simulink model "ConSys_A1"  (Simulink 8.3)
settings: Solver=ode3  StartTime=0.0  StopTime=Time(end)  FixedStep=Ts  RelTol=1e-3
values from neighbouring files (symbols this model uses):
  d = r*h    (= 1.6)    [StartUp_A1.m]
  d0 = d*h    (= 0.0032)    [StartUp_A1.m]
  h = 0.002    [StartUp_A1.m]
  Ka = diag([ 3  20  20  150  355  520])    [StartUp_A1.m]
  Kd = diag([ 3   5  25  100   15 1050])    [StartUp_A1.m]
  Ki = diag([35 555 810 7410 1850 5815])    [StartUp_A1.m]
  Kp = diag([55 180 350 1960  680 4450])    [StartUp_A1.m]
  r = 800    [StartUp_A1.m]
  TD = ss(Atd,Btd,Ctd,Dtd,Ts)    [StartUp_A1.m]
  Ts = 1/200    (= 0.005)    [StartUp_A1.m]
undefined symbols (not defined in the file or in its folder): DiscIntNeverNeededParam
undefined symbols (not defined in the file): ADAMS_cwd, ADAMS_exec, ADAMS_host, ADAMS_init, ADAMS_inputs, ADAMS_outputs, ADAMS_prefix, ADAMS_static, ADAMS_sysdir
libraries: cstblocks x6
(part 8 of 9)

== matlab function A2/MATLAB Function 5 ==
  data: q input double; V5 output double; dq input double
function V5 = V5(q,dq)
%#codegen
Th1=q(1,1); Th2=q(2,1); Th3=q(3,1); Th4=q(4,1); Th5=q(5,1); Th6=q(6,1);
dTh1=dq(1); dTh2=dq(2); dTh3=dq(3); dTh4=dq(4); dTh5=dq(5); dTh6=dq(6);
%---------------------------
V511=(0.5*(sin(Th2 + Th3)*cos(Th5) + cos(Th2 + Th3)*cos(Th4)*sin(Th5))*(4.0e-6*cos(Th6)*(sin(Th2 + Th3)*cos(Th5) + cos(Th2 + Th3)*cos(Th4)*sin(Th5)) + 0.000116*sin(Th2 + Th3)*sin(Th5) - 0.000116*cos(Th2 + Th3)*cos(Th4)*cos(Th5)) - 0.5*(cos(Th6)*(sin(Th2 + Th3)*sin(Th5) - 1.0*cos(Th2 + Th3)*cos(Th4)*cos(Th5)) + cos(Th2 + Th3)*sin(Th4)*sin(Th6))*(0.001043*cos(Th6)*(sin(Th2 + Th3)*cos(Th5) + cos(Th2 + Th3)*cos(Th4)*sin(Th5)) + 4.0e-6*sin(Th2 + Th3)*sin(Th5) - 4.0e-6*cos(Th2 + Th3)*cos(Th4)*cos(Th5)) - 0.5*(sin(Th2 + Th3)*sin(Th5) - 1.0*cos(Th2 + Th3)*cos(Th4)*cos(Th5))*(4.0e-6*cos(Th6)*(sin(Th2 + Th3)*sin(Th5) - 1.0*cos(Th2 + Th3)*cos(Th4)*cos(Th5)) - 0.000116*sin(Th2 + Th3)*cos(Th5) - 0.000116*cos(Th2 + Th3)*cos(Th4)*sin(Th5) + 4.0e-6*cos(Th2 + Th3)*sin(Th4)*sin(Th6)) - 1.0*(0.000115*cos(Th6)*(sin(Th5)*(sin(Th1)*sin(Th4) - 1.0*sin(Th2 + Th3)*cos(Th1)*cos(Th4)) + cos(Th2 + Th3)*cos(Th1)*cos(Th5)) + 0.02603*cos(Th5)*(sin(Th1)*sin(Th4) - 1.0*sin(Th2 + Th3)*cos(Th1)*cos(Th4)) - 0.02603*cos(Th2 + Th3)*cos(Th1)*sin(Th5))*(0.07*cos(Th1) + 0.05206*sin(Th5)*(sin(Th1)*sin(Th4) - 1.0*sin(Th2 + Th3)*cos(Th1)*cos(Th4)) + 0.126*cos(Th2 + Th3)*cos(Th1) - 0.00023*sin(Th6)*(cos(Th4)*sin(Th1) + sin(Th2 + Th3)*cos(Th1)*sin(Th4)) - 0.36*cos(Th1)*sin(Th2) - 0.00023*cos(Th6)*(cos(Th5)*(sin(Th1)*sin(Th4) - 1.0*sin(Th2 + Th3)*cos(Th1)*cos(Th4)) - 1.0*cos(Th2 + Th3)*cos(Th1)*sin(Th5)) + 0.05206*cos(Th2 + Th3)*cos(Th1)*cos(Th5) + 0.254*cos(Th1)*cos(Th2)*cos(Th3) - 0.254*cos(Th1)*sin(Th2)*sin(Th3)) + (0.00152*cos(Th5)*(cos(Th1)*sin(Th4) + sin(Th2 + Th3)*cos(Th4)*sin(Th1)) + 0.00002*sin(Th5)*(cos(Th1)*sin(Th4) + sin(Th2 + Th3)*cos(Th4)*sin(Th1)) - 0.00002*cos(Th2 + Th3)*cos(Th5)*sin(Th1) + 0.00152*cos(Th2 + Th3)*sin(Th1)*sin(Th5))*(0.00002*cos(Th5)*(cos(Th1)*sin(Th4) + sin(Th2 + Th3)*cos(Th4)*sin(Th1)) - 0.126*cos(Th2 + Th3)*sin(Th1) - 0.07*sin(Th1) - 0.00152*sin(Th5)*(cos(Th1)*sin(Th4) + sin(Th2 + Th3)*cos(Th4)*sin(Th1)) - 0.00062*cos(Th1)*cos(Th4) + 0.36*sin(Th1)*sin(Th2) + 0.00152*cos(Th2 + Th3)*cos(Th5)*sin(Th1) + 0.00002*cos(Th2 + Th3)*sin(Th1)*sin(Th5) + 0.00062*sin(Th2 + Th3)*sin(Th1)*sin(Th4) - 0.254*cos(Th2)*cos(Th3)*sin(Th1) + 0.254*sin(Th1)*sin(Th2)*sin(Th3)) - 1.0*(0.00152*cos(Th5)*(sin(Th1)*sin(Th4) - 1.0*sin(Th2 + Th3)*cos(Th1)*cos(Th4)) + 0.00002*sin(Th5)*(sin(Th1)*sin(Th4) - 1.0*sin(Th2 + Th3)*cos(Th1)*cos(Th4)) + 0.00002*cos(Th2 + Th3)*cos(Th1)*cos(Th5) - 0.00152*cos(Th2 + Th3)*cos(Th1)*sin(Th5))*(0.00152*sin(Th5)*(sin(Th1)*sin(Th4) - 1.0*sin(Th2 + Th3)*cos(Th1)*cos(Th4)) - 0.00002*cos(Th5)*(sin(Th1)*sin(Th4) - 1.0*sin(Th2 + Th3)*cos(Th1)*cos(Th4)) - 0.07*cos(Th1) - 0.126*cos(Th2 + Th3)*cos(Th1) + 0.36*cos(Th1)*sin(Th2) + 0.00062*cos(Th4)*sin(Th1) + 0.00152*cos(Th2 + Th3)*cos(Th1)*cos(Th5) + 0.00002*cos(Th2 + Th3)*cos(Th1)*sin(Th5) + 0.00062*sin(Th2 + Th3)*cos(Th1)*sin(Th4) - 0.254*cos(Th1)*cos(Th2)*cos(Th3) + 0.254*cos(Th1)*sin(Th2)*sin(Th3)) + (0.000115*cos(Th6)*(sin(Th5)*(cos(Th1)*sin(Th4) + sin(Th2 + Th3)*cos(Th4)*sin(Th1)) - 1.0*cos(Th2 + Th3)*cos(Th5)*sin(Th1)) + 0.02603*cos(Th5)*(cos(Th1)*sin(Th4) + sin(Th2 + Th3)*cos(Th4)*sin(Th1)) + 0.02603*cos(Th2 + Th3)*sin(Th1)*sin(Th5))*(0.07*sin(Th1) + 0.00023*sin(Th6)*(cos(Th1)*cos(Th4) - 1.0*sin(Th2 + Th3)*sin(Th1)*sin(Th4)) + 0.00023*cos(Th6)*(cos(Th5)*(cos(Th1)*sin(Th4) + sin(Th2 + Th3)*cos(Th4)*sin(Th1)) + cos(Th2 + Th3)*sin(Th1)*sin(Th5)) + 0.126*cos(Th2 + Th3)*sin(Th1) - 0.05206*sin(Th5)*(cos(Th1)*sin(Th4) + sin(Th2 + Th3)*cos(Th4)*sin(Th1)) - 0.36*sin(Th1)*sin(Th2) + 0.05206*cos(Th2 + Th3)*cos(Th5)*sin(Th1) + 0.254*cos(Th2)*cos(Th3)*sin(Th1) - 0.254*sin(Th1)*sin(Th2)*sin(Th3)) - 0.5*cos(Th6)*(sin(Th2 + Th3)*cos(Th5) + cos(Th2 + Th3)*cos(Th4)*sin(Th5))*(0.001043*cos(Th6)*(sin(Th2 + Th3)*sin(Th5) - 1.0*cos(Th2 + Th3)*cos(Th4)*cos(Th5)) - 4.0e-6*sin(Th2 + Th3)*cos(Th5) - 4.0e-6*cos(Th2 + Th3)*cos(Th4)*sin(Th5) + 0.001043*cos(Th2 + Th3)*sin(Th4)*sin(Th6)) - 0.5*sin(Th6)*(sin(Th2 + Th3)*cos(Th5) + cos(Th2 + Th3)*cos(Th4)*sin(Th5))*(0.00104*sin(Th6)*(sin(Th2 + Th3)*sin(Th5) - 1.0*cos(Th2 + Th3)*cos(Th4)*cos(Th5)) - 0.00104*cos(Th2 + Th3)*cos(Th6)*sin(Th4)) - 0.004409*sin(Th2 + Th3)^2*cos(Th5)*sin(Th5) - 0.00052*sin(Th6)*(sin(Th2 + Th3)*cos(Th5) + cos(Th2 + Th3)*cos(Th4)*sin(Th5))*(sin(Th6)*(sin(Th2 + Th3)*sin(Th5) - 1.0*cos(Th2 + Th3)*cos(Th4)*cos(Th5)) - 1.0*cos(Th2 + Th3)*cos(Th6)*sin(Th4)) + 0.004409*cos(Th2 + Th3)*sin(Th2 + Th3)*cos(Th4)*cos(Th5)^2 - 0.004409*cos(Th2 + Th3)*sin(Th2 + Th3)*cos(Th4)*sin(Th5)^2 + 0.00004*cos(Th2 + Th3)^2*cos(Th4)*cos(Th5)*sin(Th4) + 0.004409*cos(Th2 + Th3)^2*cos(Th4)^2*cos(Th5)*sin(Th5) - 0.00004*cos(Th2 + Th3)*sin(Th2 + Th3)*sin(Th4)*sin(Th5))*dTh1*dTh1;
V512=(0.000058586*cos(Th2)*cos(Th3)*cos(Th5) - 1.86e-8*cos(Th2)*cos(Th3)*sin(Th5) + 0.013235*cos(Th2)*cos(Th5)*sin(Th4) + 0.0042472*cos(Th2)*sin(Th3)*sin(Th4) + 0.0042472*cos(Th3)*sin(Th2)*sin(Th4) - 0.000058586*cos(Th5)*sin(Th2)*sin(Th3) - 0.0000108*cos(Th2)*sin(Th4)*sin(Th5) + 1.86e-8*sin(Th2)*sin(Th3)*sin(Th5) + 3.04e-8*cos(Th2)*cos(Th3)*cos(Th4)*sin(Th4) - 6.2e-9*cos(Th2)*cos(Th4)*cos(Th5)*sin(Th3) - 6.2e-9*cos(Th3)*cos(Th4)*cos(Th5)*sin(Th2) + 0.00001498*cos(Th2)*cos(Th3)*cos(Th5)*sin(Th6) - 0.000019529*cos(Th2)*cos(Th4)*sin(Th3)*sin(Th5) + 0.013971*cos(Th2)*cos(Th5)*sin(Th3)*sin(Th4) - 0.000019529*cos(Th3)*cos(Th4)*sin(Th2)*sin(Th5) + 0.013971*cos(Th3)*cos(Th5)*sin(Th2)*sin(Th4) + 0.0000621*cos(Th2)*cos(Th6)*sin(Th4)*sin(Th5) - 3.04e-8*cos(Th4)*sin(Th2)*sin(Th3)*sin(Th4) - 0.0000114*cos(Th2)*sin(Th3)*sin(Th4)*sin(Th5) - 0.0000114*cos(Th3)*sin(Th2)*sin(Th4)*sin(Th5) - 0.00001498*cos(Th5)*sin(Th2)*sin(Th3)*sin(Th6) - 0.000039058*cos(Th2)*cos(Th3)*cos(Th4)^2*cos(Th5) + 1.24e-8*cos(Th2)*cos(Th3)*cos(Th4)^2*sin(Th5) + 0.0066904*cos(Th2)*cos(Th5)^2*sin(Th3)*sin(Th4) + 0.0066904*cos(Th3)*cos(Th5)^2*sin(Th2)*sin(Th4) + 0.000039058*cos(Th4)^2*cos(Th5)*sin(Th2)*sin(Th3) - 4.4603e-6*cos(Th2)*cos(Th6)^2*sin(Th3)*sin(Th4) - 4.4603e-6*cos(Th3)*cos(Th6)^2*sin(Th2)*sin(Th4) - 1.24e-8*cos(Th4)^2*sin(Th2)*sin(Th3)*sin(Th5) + 9.9869e-6*cos(Th2)*cos(Th3)*cos(Th4)*cos(Th6)*sin(Th4) - 4.4603e-6*cos(Th2)*cos(Th3)*cos(Th6)*sin(Th5)*sin(Th6) + 6.08e-8*cos(Th2)*cos(Th5)*sin(Th3)*sin(Th4)*sin(Th5) + 6.08e-8*cos(Th3)*cos(Th5)*sin(Th2)*sin(Th4)*sin(Th5) - 9.9869e-6*cos(Th4)*cos(Th6)*sin(Th2)*sin(Th3)*sin(Th4) - 4.9934e-6*cos(Th2)*cos(Th4)*sin(Th3)*sin(Th5)*sin(Th6) + 0.00006555*cos(Th2)*cos(Th6)*sin(Th3)*sin(Th4)*sin(Th5) - 4.9934e-6*cos(Th3)*cos(Th4)*sin(Th2)*sin(Th5)*sin(Th6) + 0.00006555*cos(Th3)*cos(Th6)*sin(Th2)*sin(Th4)*sin(Th5) + 4.4603e-6*cos(Th6)*sin(Th2)*sin(Th3)*sin(Th5)*sin(Th6) - 6.08e-8*cos(Th2)*cos(Th3)*cos(Th4)*cos(Th5)^2*sin(Th4) - 9.9869e-6*cos(Th2)*cos(Th3)*cos(Th4)^2*cos(Th5)*sin(Th6) + 6.08e-8*cos(Th4)*cos(Th5)^2*sin(Th2)*sin(Th3)*sin(Th4) + 9.9869e-6*cos(Th4)^2*cos(Th5)*sin(Th2)*sin(Th3)*sin(Th6) + 2.9736e-6*cos(Th2)*cos(Th5)^2*cos(Th6)^2*sin(Th3)*sin(Th4) + 2.9736e-6*cos(Th3)*cos(Th5)^2*cos(Th6)^2*sin(Th2)*sin(Th4) - 0.000019974*cos(Th2)*cos(Th3)*cos(Th4)*cos(Th5)^2*cos(Th6)*sin(Th4) + 2.9736e-6*cos(Th2)*cos(Th3)*cos(Th4)^2*cos(Th6)*sin(Th5)*sin(Th6) + 0.000019974*cos(Th4)*cos(Th5)^2*cos(Th6)*sin(Th2)*sin(Th3)*sin(Th4) - 2.9736e-6*cos(Th4)^2*cos(Th6)*sin(Th2)*sin(Th3)*sin(Th5)*sin(Th6) + 0.0066904*cos(Th2)*cos(Th3)*cos(Th4)*cos(Th5)*sin(Th4)*sin(Th5) - 1.4868e-6*cos(Th2)*cos(Th4)*cos(Th5)*cos(Th6)*sin(Th3)*sin(Th6) - 1.4868e-6*cos(Th3)*cos(Th4)*cos(Th5)*cos(Th6)*sin(Th2)*sin(Th6) + 0.000019974*cos(Th2)*cos(Th5)*cos(Th6)*sin(Th3)*sin(Th4)*sin(Th5) + 0.000019974*cos(Th3)*cos(Th5)*cos(Th6)*sin(Th2)*sin(Th4)*sin(Th5) - 0.0066904*cos(Th4)*cos(Th5)*sin(Th2)*sin(Th3)*sin(Th4)*sin(Th5) - 2.9736e-6*cos(Th4)*cos(Th5)*cos(Th6)^2*sin(Th2)*sin(Th3)*sin(Th4)*sin(Th5) + 2.9736e-6*cos(Th2)*cos(Th3)*cos(Th4)*cos(Th5)*cos(Th6)^2*sin(Th4)*sin(Th5))*dTh1*dTh2;
V513=(0.000058586*cos(Th2)*cos(Th3)*cos(Th5) - 1.86e-8*cos(Th2)*cos(Th3)*sin(Th5) + 0.0042472*cos(Th2)*sin(Th3)*sin(Th4) + 0.0042472*cos(Th3)*sin(Th2)*sin(Th4) - 0.000058586*cos(Th5)*sin(Th2)*sin(Th3) + 1.86e-8*sin(Th2)*sin(Th3)*sin(Th5) + 3.04e-8*cos(Th2)*cos(Th3)*cos(Th4)*sin(Th4) - 6.2e-9*cos(Th2)*cos(Th4)*cos(Th5)*sin(Th3) - 6.2e-9*cos(Th3)*cos(Th4)*cos(Th5)*sin(Th2) + 0.00001498*cos(Th2)*cos(Th3)*cos(Th5)*sin(Th6) - 0.000019529*cos(Th2)*cos(Th4)*sin(Th3)*sin(Th5) + 0.013971*cos(Th2)*cos(Th5)*sin(Th3)*sin(Th4) - 0.000019529*cos(Th3)*cos(Th4)*sin(Th2)*sin(Th5) + 0.013971*cos(Th3)*cos(Th5)*sin(Th2)*sin(Th4) - 3.04e-8*cos(Th4)*sin(Th2)*sin(Th3)*sin(Th4) - 0.0000114*cos(Th2)*sin(Th3)*sin(Th4)*sin(Th5) - 0.0000114*cos(Th3)*sin(Th2)*sin(Th4)*sin(Th5) - 0.00001498*cos(Th5)*sin(Th2)*sin(Th3)*sin(Th6) - 0.000039058*cos(Th2)*cos(Th3)*cos(Th4)^2*cos(Th5) + 1.24e-8*cos(Th2)*cos(Th3)*cos(Th4)^2*sin(Th5) + 0.0066904*cos(Th2)*cos(Th5)^2*sin(Th3)*sin(Th4) + 0.0066904*cos(Th3)*cos(Th5)^2*sin(Th2)*sin(Th4) + 0.000039058*cos(Th4)^2*cos(Th5)*sin(Th2)*sin(Th3) - 4.4603e-6*cos(Th2)*cos(Th6)^2*sin(Th3)*sin(Th4) - 4.4603e-6*cos(Th3)*cos(Th6)^2*sin(Th2)*sin(Th4) - 1.24e-8*cos(Th4)^2*sin(Th2)*sin(Th3)*sin(Th5) + 9.9869e-6*cos(Th2)*cos(Th3)*cos(Th4)*cos(Th6)*sin(Th4) - 4.4603e-6*cos(Th2)*cos(Th3)*cos(Th6)*sin(Th5)*sin(Th6) + 6.08e-8*cos(Th2)*cos(Th5)*sin(Th3)*sin(Th4)*sin(Th5) + 6.08e-8*cos(Th3)*cos(Th5)*sin(Th2)*sin(Th4)*sin(Th5) - 9.9869e-6*cos(Th4)*cos(Th6)*sin(Th2)*sin(Th3)*sin(Th4) - 4.9934e-6*cos(Th2)*cos(Th4)*sin(Th3)*sin(Th5)*sin(Th6) + 0.00006555*cos(Th2)*cos(Th6)*sin(Th3)*sin(Th4)*sin(Th5) - 4.9934e-6*cos(Th3)*cos(Th4)*sin(Th2)*sin(Th5)*sin(Th6) + 0.00006555*cos(Th3)*cos(Th6)*sin(Th2)*sin(Th4)*sin(Th5) + 4.4603e-6*cos(Th6)*sin(Th2)*sin(Th3)*sin(Th5)*sin(Th6) - 6.08e-8*cos(Th2)*cos(Th3)*cos(Th4)*cos(Th5)^2*sin(Th4) - 9.9869e-6*cos(Th2)*cos(Th3)*cos(Th4)^2*cos(Th5)*sin(Th6) + 6.08e-8*cos(Th4)*cos(Th5)^2*sin(Th2)*sin(Th3)*sin(Th4) + 9.9869e-6*cos(Th4)^2*cos(Th5)*sin(Th2)*sin(Th3)*sin(Th6) + 2.9736e-6*cos(Th2)*cos(Th5)^2*cos(Th6)^2*sin(Th3)*sin(Th4) + 2.9736e-6*cos(Th3)*cos(Th5)^2*cos(Th6)^2*sin(Th2)*sin(Th4) - 0.000019974*cos(Th2)*cos(Th3)*cos(Th4)*cos(Th5)^2*cos(Th6)*sin(Th4) + 2.9736e-6*cos(Th2)*cos(Th3)*cos(Th4)^2*cos(Th6)*sin(Th5)*sin(Th6) + 0.000019974*cos(Th4)*cos(Th5)^2*cos(Th6)*sin(Th2)*sin(Th3)*sin(Th4) - 2.9736e-6*cos(Th4)^2*cos(Th6)*sin(Th2)*sin(Th3)*sin(Th5)*sin(Th6) + 0.0066904*cos(Th2)*cos(Th3)*cos(Th4)*cos(Th5)*sin(Th4)*sin(Th5) - 1.4868e-6*cos(Th2)*cos(Th4)*cos(Th5)*cos(Th6)*sin(Th3)*sin(Th6) - 1.4868e-6*cos(Th3)*cos(Th4)*cos(Th5)*cos(Th6)*sin(Th2)*sin(Th6) + 0.000019974*cos(Th2)*cos(Th5)*cos(Th6)*sin(Th3)*sin(Th4)*sin(Th5) + 0.000019974*cos(Th3)*cos(Th5)*cos(Th6)*sin(Th2)*sin(Th4)*sin(Th5) - 0.0066904*cos(Th4)*cos(Th5)*sin(Th2)*sin(Th3)*sin(Th4)*sin(Th5) - 2.9736e-6*cos(Th4)*cos(Th5)*cos(Th6)^2*sin(Th2)*sin(Th3)*sin(Th4)*sin(Th5) + 2.9736e-6*cos(Th2)*cos(Th3)*cos(Th4)*cos(Th5)*cos(Th6)^2*sin(Th4)*sin(Th5))*dTh1*dTh3;
V514=(7.0e-7*cos(Th4)*sin(Th5) - 3.04e-8*cos(Th2)*sin(Th3) - 3.04e-8*cos(Th3)*sin(Th2) - 0.00085785*cos(Th4)*cos(Th5) - 0.010938*cos(Th2)*cos(Th3)*cos(Th4) - 9.9869e-6*cos(Th2)*cos(Th6)*sin(Th3) - 9.9869e-6*cos(Th3)*cos(Th6)*sin(Th2) + 0.0044118*cos(Th4)*cos(Th5)*sin(Th2) - 4.025e-6*cos(Th4)*cos(Th6)*sin(Th5) + 0.010938*cos(Th4)*sin(Th2)*sin(Th3) - 3.6e-6*cos(Th4)*sin(Th2)*sin(Th5) + 6.08e-8*cos(Th2)*cos(Th5)^2*sin(Th3) + 6.08e-8*cos(Th3)*cos(Th5)^2*sin(Th2) - 0.0046569*cos(Th2)*cos(Th3)*cos(Th4)*cos(Th5) + 3.8e-6*cos(Th2)*cos(Th3)*cos(Th4)*sin(Th5) - 1.86e-8*cos(Th2)*cos(Th3)*cos(Th5)*sin(Th4) - 0.000058586*cos(Th2)*cos(Th3)*sin(Th4)*sin(Th5) + 0.0046569*cos(Th4)*cos(Th5)*sin(Th2)*sin(Th3) - 0.0066904*cos(Th2)*cos(Th5)*sin(Th3)*sin(Th5) - 0.0066904*cos(Th3)*cos(Th5)*sin(Th2)*sin(Th5) + 0.0000207*cos(Th4)*cos(Th6)*sin(Th2)*sin(Th5) - 3.8e-6*cos(Th4)*sin(Th2)*sin(Th3)*sin(Th5) + 1.86e-8*cos(Th5)*sin(Th2)*sin(Th3)*sin(Th4) + 0.000058586*sin(Th2)*sin(Th3)*sin(Th4)*sin(Th5) + 0.0066904*cos(Th2)*cos(Th3)*cos(Th4)*cos(Th5)^2 + 1.4868e-6*cos(Th2)*cos(Th3)*cos(Th4)*cos(Th6)^2 + 0.000019974*cos(Th2)*cos(Th5)^2*cos(Th6)*sin(Th3) + 0.000019974*cos(Th3)*cos(Th5)^2*cos(Th6)*sin(Th2) - 0.0066904*cos(Th4)*cos(Th5)^2*sin(Th2)*sin(Th3) - 1.4868e-6*cos(Th4)*cos(Th6)^2*sin(Th2)*sin(Th3) + 6.08e-8*cos(Th2)*cos(Th3)*cos(Th4)*cos(Th5)*sin(Th5) - 0.00002185*cos(Th2)*cos(Th3)*cos(Th4)*cos(Th6)*sin(Th5) - 6.08e-8*cos(Th4)*cos(Th5)*sin(Th2)*sin(Th3)*sin(Th5) - 0.00001498*cos(Th2)*cos(Th3)*sin(Th4)*sin(Th5)*sin(Th6) + 0.00002185*cos(Th4)*cos(Th6)*sin(Th2)*sin(Th3)*sin(Th5) + 0.00001498*sin(Th2)*sin(Th3)*sin(Th4)*sin(Th5)*sin(Th6) - 2.9736e-6*cos(Th2)*cos(Th5)*cos(Th6)^2*sin(Th3)*sin(Th5) - 2.9736e-6*cos(Th3)*cos(Th5)*cos(Th6)^2*sin(Th2)*sin(Th5) + 2.9736e-6*cos(Th2)*cos(Th3)*cos(Th4)*cos(Th5)^2*cos(Th6)^2 - 2.9736e-6*cos(Th4)*cos(Th5)^2*cos(Th6)^2*sin(Th2)*sin(Th3) + 0.000019974*cos(Th2)*cos(Th3)*cos(Th4)*cos(Th5)*cos(Th6)*sin(Th5) - 4.4603e-6*cos(Th2)*cos(Th3)*cos(Th5)*cos(Th6)*sin(Th4)*sin(Th6) - 0.000019974*cos(Th4)*cos(Th5)*cos(Th6)*sin(Th2)*sin(Th3)*sin(Th5) + 4.4603e-6*cos(Th5)*cos(Th6)*sin(Th2)*sin(Th3)*sin(Th4)*sin(Th6))*dTh1*dTh4;
V515=(7.0e-7*cos(Th5)*sin(Th4) + 0.00085785*sin(Th4)*sin(Th5) - 6.2e-9*cos(Th2)*cos(Th5)*sin(Th3) - 6.2e-9*cos(Th3)*cos(Th5)*sin(Th2) - 4.025e-6*cos(Th5)*cos(Th6)*sin(Th4) - 0.000019529*cos(Th2)*sin(Th3)*sin(Th5) - 0.000019529*cos(Th3)*sin(Th2)*sin(Th5) - 3.6e-6*cos(Th5)*sin(Th2)*sin(Th4) - 0.0044118*sin(Th2)*sin(Th4)*sin(Th5) + 0.000019529*cos(Th2)*cos(Th3)*cos(Th4)*cos(Th5) - 6.2e-9*cos(Th2)*cos(Th3)*cos(Th4)*sin(Th5) + 3.8e-6*cos(Th2)*cos(Th3)*cos(Th5)*sin(Th4) + 0.0046569*cos(Th2)*cos(Th3)*sin(Th4)*sin(Th5) - 0.000019529*cos(Th4)*cos(Th5)*sin(Th2)*sin(Th3) + 0.0000207*cos(Th5)*cos(Th6)*sin(Th2)*sin(Th4) + 6.2e-9*cos(Th4)*sin(Th2)*sin(Th3)*sin(Th5) - 3.8e-6*cos(Th5)*sin(Th2)*sin(Th3)*sin(Th4) - 4.9934e-6*cos(Th2)*sin(Th3)*sin(Th5)*sin(Th6) - 4.9934e-6*cos(Th3)*sin(Th2)*sin(Th5)*sin(Th6) - 0.0046569*sin(Th2)*sin(Th3)*sin(Th4)*sin(Th5) + 4.9934e-6*cos(Th2)*cos(Th3)*cos(Th4)*cos(Th5)*sin(Th6) - 0.00002185*cos(Th2)*cos(Th3)*cos(Th5)*cos(Th6)*sin(Th4) - 1.4868e-6*cos(Th2)*cos(Th5)*cos(Th6)*sin(Th3)*sin(Th6) - 1.4868e-6*cos(Th3)*cos(Th5)*cos(Th6)*sin(Th2)*sin(Th6) - 4.9934e-6*cos(Th4)*cos(Th5)*sin(Th2)*sin(Th3)*sin(Th6) + 0.00002185*cos(Th5)*cos(Th6)*sin(Th2)*sin(Th3)*sin(Th4) - 1.4868e-6*cos(Th2)*cos(Th3)*cos(Th4)*cos(Th6)*sin(Th5)*sin(Th6) + 1.4868e-6*cos(Th4)*cos(Th6)*sin(Th2)*sin(Th3)*sin(Th5)*sin(Th6))*dTh1*dTh5;
V516=(0.000060987*cos(Th2)*sin(Th3)*sin(Th5) + 0.000060987*cos(Th3)*sin(Th2)*sin(Th5) + 4.025e-6*sin(Th4)*sin(Th5)*sin(Th6) - 0.000060987*cos(Th2)*cos(Th3)*cos(Th4)*cos(Th5) + 0.00001498*cos(Th2)*cos(Th5)*cos(Th6)*sin(Th3) + 0.00001498*cos(Th3)*cos(Th5)*cos(Th6)*sin(Th2) + 0.000060987*cos(Th4)*cos(Th5)*sin(Th2)*sin(Th3) - 0.0000207*sin(Th2)*sin(Th4)*sin(Th5)*sin(Th6) - 5.9471e-6*cos(Th2)*cos(Th6)^2*sin(Th3)*sin(Th5) - 5.9471e-6*cos(Th3)*cos(Th6)^2*sin(Th2)*sin(Th5) + 0.00001498*cos(Th2)*cos(Th3)*cos(Th4)*cos(Th6)*sin(Th5) - 5.9471e-6*cos(Th2)*cos(Th3)*cos(Th6)*sin(Th4)*sin(Th6) + 0.00002185*cos(Th2)*cos(Th3)*sin(Th4)*sin(Th5)*sin(Th6) - 0.00001498*cos(Th4)*cos(Th6)*sin(Th2)*sin(Th3)*sin(Th5) + 5.9471e-6*cos(Th6)*sin(Th2)*sin(Th3)*sin(Th4)*sin(Th6) - 0.00002185*sin(Th2)*sin(Th3)*sin(Th4)*sin(Th5)*sin(Th6) + 5.9471e-6*cos(Th2)*cos(Th3)*cos(Th4)*cos(Th5)*cos(Th6)^2 - 5.9471e-6*cos(Th4)*cos(Th5)*cos(Th6)^2*sin(Th2)*sin(Th3))*dTh1*dTh6;
%---------------------------
V521=(0.00002*cos(Th2 + Th3)*cos(Th5) - 0.0026665*sin(Th2 + Th3)*sin(Th4) + 6.2e-9*sin(Th2 + Th3)*cos(Th4)*cos(Th5) + 2.0e-6*cos(Th2 + Th3)*cos(Th5)*sin(Th6) + 0.000019529*sin(Th2 + Th3)*cos(Th4)*sin(Th5) + 0.0015441*sin(Th2 + Th3)*cos(Th5)*sin(Th4) - 1.26e-6*sin(Th2 + Th3)*sin(Th4)*sin(Th5) + 0.0044118*cos(Th2)*cos(Th5)*sin(Th4) - 0.000039529*cos(Th2 + Th3)*cos(Th4)^2*cos(Th5) - 3.6e-6*cos(Th2)*sin(Th4)*sin(Th5) - 4.712e-7*cos(Th2 + Th3)*cos(Th5)*sin(Th4)^2 + 6.2e-9*cos(Th2 + Th3)*cos(Th4)^2*sin(Th5) - 6.2e-9*cos(Th2 + Th3)*sin(Th4)^2*sin(Th5) + 0.0060117*sin(Th2 + Th3)*cos(Th5)^2*sin(Th4) - 1.5e-6*sin(Th2 + Th3)*cos(Th6)^2*sin(Th4) - 0.00067872*sin(Th2 + Th3)*sin(Th4)*sin(Th5)^2 + 4.0e-6*cos(Th2 + Th3)*cos(Th4)*cos(Th6)*sin(Th4) - 1.5e-6*cos(Th2 + Th3)*cos(Th6)*sin(Th5)*sin(Th6) + 6.08e-8*sin(Th2 + Th3)*cos(Th5)*sin(Th4)*sin(Th5) + 4.9934e-6*sin(Th2 + Th3)*cos(Th4)*sin(Th5)*sin(Th6) + 7.245e-6*sin(Th2 + Th3)*cos(Th6)*sin(Th4)*sin(Th5) + 0.0031128*cos(Th2)*cos(Th5)*sin(Th3)*sin(Th4) + 0.0031128*cos(Th3)*cos(Th5)*sin(Th2)*sin(Th4) + 0.0000207*cos(Th2)*cos(Th6)*sin(Th4)*sin(Th5) - 3.04e-8*cos(Th2 + Th3)*cos(Th4)*cos(Th5)^2*sin(Th4) - 6.9935e-6*cos(Th2 + Th3)*cos(Th4)^2*cos(Th5)*sin(Th6) - 2.54e-6*cos(Th2)*sin(Th3)*sin(Th4)*sin(Th5) - 2.54e-6*cos(Th3)*sin(Th2)*sin(Th4)*sin(Th5) + 3.04e-8*cos(Th2 + Th3)*cos(Th4)*sin(Th4)*sin(Th5)^2 + 2.9935e-6*cos(Th2 + Th3)*cos(Th5)*sin(Th4)^2*sin(Th6) + 2.9868e-6*sin(Th2 + Th3)*cos(Th5)^2*cos(Th6)^2*sin(Th4) + 1.3225e-8*sin(Th2 + Th3)*cos(Th6)^2*sin(Th4)*sin(Th5)^2 - 0.000013987*cos(Th2 + Th3)*cos(Th4)*cos(Th5)^2*cos(Th6)*sin(Th4) + 0.000014605*cos(Th2)*cos(Th6)*sin(Th3)*sin(Th4)*sin(Th5) + 0.000014605*cos(Th3)*cos(Th6)*sin(Th2)*sin(Th4)*sin(Th5) + 5.9869e-6*cos(Th2 + Th3)*cos(Th4)*cos(Th6)*sin(Th4)*sin(Th5)^2 + 2.9868e-6*cos(Th2 + Th3)*cos(Th4)^2*cos(Th6)*sin(Th5)*sin(Th6) + 1.3225e-8*cos(Th2 + Th3)*cos(Th6)*sin(Th4)^2*sin(Th5)*sin(Th6) + 0.0066904*cos(Th2 + Th3)*cos(Th4)*cos(Th5)*sin(Th4)*sin(Th5) + 1.4868e-6*sin(Th2 + Th3)*cos(Th4)*cos(Th5)*cos(Th6)*sin(Th6) + 0.000019974*sin(Th2 + Th3)*cos(Th5)*cos(Th6)*sin(Th4)*sin(Th5) + 2.9736e-6*cos(Th2 + Th3)*cos(Th4)*cos(Th5)*cos(Th6)^2*sin(Th4)*sin(Th5))*dTh2*dTh1;
V522=(0.0033452*sin(2.0*Th5) + 7.6e-6*cos(Th5) + 9.9869e-6*cos(Th6) + 0.0093138*sin(Th5) - 3.04e-8*cos(Th4)^2 - 6.08e-8*cos(Th5)^2 - 9.9869e-6*cos(Th4)^2*cos(Th6) - 0.000019974*cos(Th5)^2*cos(Th6) + 6.08e-8*cos(Th4)^2*cos(Th5)^2 - 0.0000437*cos(Th5)*cos(Th6) + 7.2e-6*cos(Th5)*sin(Th3) + 0.0088236*sin(Th3)*sin(Th5) + 0.000019974*cos(Th4)^2*cos(Th5)^2*cos(Th6) - 0.0088236*cos(Th3)*cos(Th4)*cos(Th5) + 7.2e-6*cos(Th3)*cos(Th4)*sin(Th5) - 0.000039058*cos(Th4)*cos(Th5)*sin(Th4) - 0.0000414*cos(Th5)*cos(Th6)*sin(Th3) + 1.24e-8*cos(Th4)*sin(Th4)*sin(Th5) - 0.0066904*cos(Th4)^2*cos(Th5)*sin(Th5) + 2.9736e-6*cos(Th5)*cos(Th6)^2*sin(Th5) - 2.9736e-6*cos(Th4)^2*cos(Th5)*cos(Th6)^2*sin(Th5) - 0.0000414*cos(Th3)*cos(Th4)*cos(Th6)*sin(Th5) - 9.9869e-6*cos(Th4)*cos(Th5)*sin(Th4)*sin(Th6) + 2.9736e-6*cos(Th4)*cos(Th6)*sin(Th4)*sin(Th5)*sin(Th6) + 3.04e-8)*dTh2*dTh2;
V523=(0.0033452*sin(2.0*Th5) + 7.6e-6*cos(Th5) + 9.9869e-6*cos(Th6) + 0.0093138*sin(Th5) - 3.04e-8*cos(Th4)^2 - 6.08e-8*cos(Th5)^2 - 9.9869e-6*cos(Th4)^2*cos(Th6) - 0.000019974*cos(Th5)^2*cos(Th6) + 6.08e-8*cos(Th4)^2*cos(Th5)^2 - 0.0000437*cos(Th5)*cos(Th6) - 3.6e-6*cos(Th5)*sin(Th3) - 0.0044118*sin(Th3)*sin(Th5) + 0.000019974*cos(Th4)^2*cos(Th5)^2*cos(Th6) + 0.0044118*cos(Th3)*cos(Th4)*cos(Th5) - 3.6e-6*cos(Th3)*cos(Th4)*sin(Th5) - 0.000039058*cos(Th4)*cos(Th5)*sin(Th4) + 0.0000207*cos(Th5)*cos(Th6)*sin(Th3) + 1.24e-8*cos(Th4)*sin(Th4)*sin(Th5) - 0.0066904*cos(Th4)^2*cos(Th5)*sin(Th5) + 2.9736e-6*cos(Th5)*cos(Th6)^2*sin(Th5) - 2.9736e-6*cos(Th4)^2*cos(Th5)*cos(Th6)^2*sin(Th5) + 0.0000207*cos(Th3)*cos(Th4)*cos(Th6)*sin(Th5) - 9.9869e-6*cos(Th4)*cos(Th5)*sin(Th4)*sin(Th6) + 2.9736e-6*cos(Th4)*cos(Th6)*sin(Th4)*sin(Th5)*sin(Th6) + 3.04e-8)*dTh2*dTh3;
V524=(0.0066904*cos(Th5)^2*sin(Th4) - 0.010938*sin(Th4) + 1.4868e-6*cos(Th6)^2*sin(Th4) + 1.86e-8*cos(Th4)*cos(Th5) + 0.000058586*cos(Th4)*sin(Th5) - 0.0046569*cos(Th5)*sin(Th4) + 3.8e-6*sin(Th4)*sin(Th5) + 2.9736e-6*cos(Th5)^2*cos(Th6)^2*sin(Th4) - 0.0044118*cos(Th5)*sin(Th3)*sin(Th4) + 6.08e-8*cos(Th5)*sin(Th4)*sin(Th5) + 0.00001498*cos(Th4)*sin(Th5)*sin(Th6) - 0.00002185*cos(Th6)*sin(Th4)*sin(Th5) + 3.6e-6*sin(Th3)*sin(Th4)*sin(Th5) + 4.4603e-6*cos(Th4)*cos(Th5)*cos(Th6)*sin(Th6) + 0.000019974*cos(Th5)*cos(Th6)*sin(Th4)*sin(Th5) - 0.0000207*cos(Th6)*sin(Th3)*sin(Th4)*sin(Th5))*dTh2*dTh4;
V525=(0.0044118*cos(Th3)*cos(Th5) - 3.8e-6*cos(Th4)*cos(Th5) - 3.6e-6*cos(Th3)*sin(Th5) - 0.0046569*cos(Th4)*sin(Th5) + 0.000019529*cos(Th5)*sin(Th4) - 6.2e-9*sin(Th4)*sin(Th5) + 0.00002185*cos(Th4)*cos(Th5)*cos(Th6) - 3.6e-6*cos(Th4)*cos(Th5)*sin(Th3) + 0.0000207*cos(Th3)*cos(Th6)*sin(Th5) - 0.0044118*cos(Th4)*sin(Th3)*sin(Th5) + 4.9934e-6*cos(Th5)*sin(Th4)*sin(Th6) + 0.0000207*cos(Th4)*cos(Th5)*cos(Th6)*sin(Th3) - 1.4868e-6*cos(Th6)*sin(Th4)*sin(Th5)*sin(Th6))*dTh2*dTh5;
V526=(0.0000207*cos(Th3)*cos(Th5)*sin(Th6) - 0.000060987*cos(Th5)*sin(Th4) + 5.9471e-6*cos(Th4)*cos(Th6)*sin(Th6) - 0.00002185*cos(Th4)*sin(Th5)*sin(Th6) + 0.00001498*cos(Th6)*sin(Th4)*sin(Th5) + 5.9471e-6*cos(Th5)*cos(Th6)^2*sin(Th4) - 0.0000207*cos(Th4)*sin(Th3)*sin(Th5)*sin(Th6))*dTh2*dTh6;
%---------------------------
V531=(0.00002*cos(Th2 + Th3)*cos(Th5) - 0.0026665*sin(Th2 + Th3)*sin(Th4) + 6.2e-9*sin(Th2 + Th3)*cos(Th4)*cos(Th5) + 2.0e-6*cos(Th2 + Th3)*cos(Th5)*sin(Th6) + 0.000019529*sin(Th2 + Th3)*cos(Th4)*sin(Th5) + 0.0015441*sin(Th2 + Th3)*cos(Th5)*sin(Th4) - 1.26e-6*sin(Th2 + Th3)*sin(Th4)*sin(Th5) - 0.000039529*cos(Th2 + Th3)*cos(Th4)^2*cos(Th5) - 4.712e-7*cos(Th2 + Th3)*cos(Th5)*sin(Th4)^2 + 6.2e-9*cos(Th2 + Th3)*cos(Th4)^2*sin(Th5) - 6.2e-9*cos(Th2 + Th3)*sin(Th4)^2*sin(Th5) + 0.0060117*sin(Th2 + Th3)*cos(Th5)^2*sin(Th4) - 1.5e-6*sin(Th2 + Th3)*cos(Th6)^2*sin(Th4) - 0.00067872*sin(Th2 + Th3)*sin(Th4)*sin(Th5)^2 + 4.0e-6*cos(Th2 + Th3)*cos(Th4)*cos(Th6)*sin(Th4) - 1.5e-6*cos(Th2 + Th3)*cos(Th6)*sin(Th5)*sin(Th6) + 6.08e-8*sin(Th2 + Th3)*cos(Th5)*sin(Th4)*sin(Th5) + 4.9934e-6*sin(Th2 + Th3)*cos(Th4)*sin(Th5)*sin(Th6) + 7.245e-6*sin(Th2 + Th3)*cos(Th6)*sin(Th4)*sin(Th5) + 0.0031128*cos(Th2)*cos(Th5)*sin(Th3)*sin(Th4) + 0.0031128*cos(Th3)*cos(Th5)*sin(Th2)*sin(Th4) - 3.04e-8*cos(Th2 + Th3)*cos(Th4)*cos(Th5)^2*sin(Th4) - 6.9935e-6*cos(Th2 + Th3)*cos(Th4)^2*cos(Th5)*sin(Th6) - 2.54e-6*cos(Th2)*sin(Th3)*sin(Th4)*sin(Th5) - 2.54e-6*cos(Th3)*sin(Th2)*sin(Th4)*sin(Th5) + 3.04e-8*cos(Th2 + Th3)*cos(Th4)*sin(Th4)*sin(Th5)^2 + 2.9935e-6*cos(Th2 + Th3)*cos(Th5)*sin(Th4)^2*sin(Th6) + 2.9868e-6*sin(Th2 + Th3)*cos(Th5)^2*cos(Th6)^2*sin(Th4) + 1.3225e-8*sin(Th2 + Th3)*cos(Th6)^2*sin(Th4)*sin(Th5)^2 - 0.000013987*cos(Th2 + Th3)*cos(Th4)*cos(Th5)^2*cos(Th6)*sin(Th4) + 0.000014605*cos(Th2)*cos(Th6)*sin(Th3)*sin(Th4)*sin(Th5) + 0.000014605*cos(Th3)*cos(Th6)*sin(Th2)*sin(Th4)*sin(Th5) + 5.9869e-6*cos(Th2 + Th3)*cos(Th4)*cos(Th6)*sin(Th4)*sin(Th5)^2 + 2.9868e-6*cos(Th2 + Th3)*cos(Th4)^2*cos(Th6)*sin(Th5)*sin(Th6) + 1.3225e-8*cos(Th2 + Th3)*cos(Th6)*sin(Th4)^2*sin(Th5)*sin(Th6) + 0.0066904*cos(Th2 + Th3)*cos(Th4)*cos(Th5)*sin(Th4)*sin(Th5) + 1.4868e-6*sin(Th2 + Th3)*cos(Th4)*cos(Th5)*cos(Th6)*sin(Th6) + 0.000019974*sin(Th2 + Th3)*cos(Th5)*cos(Th6)*sin(Th4)*sin(Th5) + 2.9736e-6*cos(Th2 + Th3)*cos(Th4)*cos(Th5)*cos(Th6)^2*sin(Th4)*sin(Th5))*dTh3*dTh1;
V532=(0.0033452*sin(2.0*Th5) + 7.6e-6*cos(Th5) + 9.9869e-6*cos(Th6) + 0.0093138*sin(Th5) - 3.04e-8*cos(Th4)^2 - 6.08e-8*cos(Th5)^2 - 9.9869e-6*cos(Th4)^2*cos(Th6) - 0.000019974*cos(Th5)^2*cos(Th6) + 6.08e-8*cos(Th4)^2*cos(Th5)^2 - 0.0000437*cos(Th5)*cos(Th6) + 3.6e-6*cos(Th5)*sin(Th3) + 0.0044118*sin(Th3)*sin(Th5) + 0.000019974*cos(Th4)^2*cos(Th5)^2*cos(Th6) - 0.0044118*cos(Th3)*cos(Th4)*cos(Th5) + 3.6e-6*cos(Th3)*cos(Th4)*sin(Th5) - 0.000039058*cos(Th4)*cos(Th5)*sin(Th4) - 0.0000207*cos(Th5)*cos(Th6)*sin(Th3) + 1.24e-8*cos(Th4)*sin(Th4)*sin(Th5) - 0.0066904*cos(Th4)^2*cos(Th5)*sin(Th5) + 2.9736e-6*cos(Th5)*cos(Th6)^2*sin(Th5) - 2.9736e-6*cos(Th4)^2*cos(Th5)*cos(Th6)^2*sin(Th5) - 0.0000207*cos(Th3)*cos(Th4)*cos(Th6)*sin(Th5) - 9.9869e-6*cos(Th4)*cos(Th5)*sin(Th4)*sin(Th6) + 2.9736e-6*cos(Th4)*cos(Th6)*sin(Th4)*sin(Th5)*sin(Th6) + 3.04e-8)*dTh3*dTh2;
V533=(0.0033452*sin(2.0*Th5) + 7.6e-6*cos(Th5) + 9.9869e-6*cos(Th6) + 0.0093138*sin(Th5) - 3.04e-8*cos(Th4)^2 - 6.08e-8*cos(Th5)^2 - 9.9869e-6*cos(Th4)^2*cos(Th6) - 0.000019974*cos(Th5)^2*cos(Th6) + 6.08e-8*cos(Th4)^2*cos(Th5)^2 - 0.0000437*cos(Th5)*cos(Th6) + 0.000019974*cos(Th4)^2*cos(Th5)^2*cos(Th6) - 0.000039058*cos(Th4)*cos(Th5)*sin(Th4) + 1.24e-8*cos(Th4)*sin(Th4)*sin(Th5) - 0.0066904*cos(Th4)^2*cos(Th5)*sin(Th5) + 2.9736e-6*cos(Th5)*cos(Th6)^2*sin(Th5) - 2.9736e-6*cos(Th4)^2*cos(Th5)*cos(Th6)^2*sin(Th5) - 9.9869e-6*cos(Th4)*cos(Th5)*sin(Th4)*sin(Th6) + 2.9736e-6*cos(Th4)*cos(Th6)*sin(Th4)*sin(Th5)*sin(Th6) + 3.04e-8)*dTh3*dTh3;
V534=(0.0066904*cos(Th5)^2*sin(Th4) - 0.010938*sin(Th4) + 1.4868e-6*cos(Th6)^2*sin(Th4) + 1.86e-8*cos(Th4)*cos(Th5) + 0.000058586*cos(Th4)*sin(Th5) - 0.0046569*cos(Th5)*sin(Th4) + 3.8e-6*sin(Th4)*sin(Th5) + 2.9736e-6*cos(Th5)^2*cos(Th6)^2*sin(Th4) + 6.08e-8*cos(Th5)*sin(Th4)*sin(Th5) + 0.00001498*cos(Th4)*sin(Th5)*sin(Th6) - 0.00002185*cos(Th6)*sin(Th4)*sin(Th5) + 4.4603e-6*cos(Th4)*cos(Th5)*cos(Th6)*sin(Th6) + 0.000019974*cos(Th5)*cos(Th6)*sin(Th4)*sin(Th5))*dTh3*dTh4;
V535=(0.000019529*cos(Th5)*sin(Th4) - 0.0046569*cos(Th4)*sin(Th5) - 3.8e-6*cos(Th4)*cos(Th5) - 6.2e-9*sin(Th4)*sin(Th5) + 0.00002185*cos(Th4)*cos(Th5)*cos(Th6) + 4.9934e-6*cos(Th5)*sin(Th4)*sin(Th6) - 1.4868e-6*cos(Th6)*sin(Th4)*sin(Th5)*sin(Th6))*dTh3*dTh5;
V536=(5.9471e-6*cos(Th4)*cos(Th6)*sin(Th6) - 0.000060987*cos(Th5)*sin(Th4) - 0.00002185*cos(Th4)*sin(Th5)*sin(Th6) + 0.00001498*cos(Th6)*sin(Th4)*sin(Th5) + 5.9471e-6*cos(Th5)*cos(Th6)^2*sin(Th4))*dTh3*dTh6;
%---------------------------
V541=(0.00085785*cos(Th4)*cos(Th5) - 3.04e-8*cos(Th2)*sin(Th3) - 3.04e-8*cos(Th3)*sin(Th2) - 7.0e-7*cos(Th4)*sin(Th5) - 0.0033452*cos(Th2)*cos(Th3)*cos(Th4) - 9.9869e-6*cos(Th2)*cos(Th6)*sin(Th3) - 9.9869e-6*cos(Th3)*cos(Th6)*sin(Th2) - 0.0044118*cos(Th4)*cos(Th5)*sin(Th2) + 4.025e-6*cos(Th4)*cos(Th6)*sin(Th5) + 0.0033452*cos(Th4)*sin(Th2)*sin(Th3) + 3.6e-6*cos(Th4)*sin(Th2)*sin(Th5) + 6.08e-8*cos(Th2)*cos(Th5)^2*sin(Th3) + 6.08e-8*cos(Th3)*cos(Th5)^2*sin(Th2) + 0.0046569*cos(Th2)*cos(Th3)*cos(Th4)*cos(Th5) - 3.8e-6*cos(Th2)*cos(Th3)*cos(Th4)*sin(Th5) - 6.2e-9*cos(Th2)*cos(Th3)*cos(Th5)*sin(Th4) - 0.000019529*cos(Th2)*cos(Th3)*sin(Th4)*sin(Th5) - 0.0046569*cos(Th4)*cos(Th5)*sin(Th2)*sin(Th3) - 0.0066904*cos(Th2)*cos(Th5)*sin(Th3)*sin(Th5) - 0.0066904*cos(Th3)*cos(Th5)*sin(Th2)*sin(Th5) - 0.0000207*cos(Th4)*cos(Th6)*sin(Th2)*sin(Th5) + 3.8e-6*cos(Th4)*sin(Th2)*sin(Th3)*sin(Th5) + 6.2e-9*cos(Th5)*sin(Th2)*sin(Th3)*sin(Th4) + 0.000019529*sin(Th2)*sin(Th3)*sin(Th4)*sin(Th5) + 0.0066904*cos(Th2)*cos(Th3)*cos(Th4)*cos(Th5)^2 - 1.4868e-6*cos(Th2)*cos(Th3)*cos(Th4)*cos(Th6)^2 + 0.000019974*cos(Th2)*cos(Th5)^2*cos(Th6)*sin(Th3) + 0.000019974*cos(Th3)*cos(Th5)^2*cos(Th6)*sin(Th2) - 0.0066904*cos(Th4)*cos(Th5)^2*sin(Th2)*sin(Th3) + 1.4868e-6*cos(Th4)*cos(Th6)^2*sin(Th2)*sin(Th3) + 6.08e-8*cos(Th2)*cos(Th3)*cos(Th4)*cos(Th5)*sin(Th5) + 0.00002185*cos(Th2)*cos(Th3)*cos(Th4)*cos(Th6)*sin(Th5) - 6.08e-8*cos(Th4)*cos(Th5)*sin(Th2)*sin(Th3)*sin(Th5) - 4.9934e-6*cos(Th2)*cos(Th3)*sin(Th4)*sin(Th5)*sin(Th6) - 0.00002185*cos(Th4)*cos(Th6)*sin(Th2)*sin(Th3)*sin(Th5) + 4.9934e-6*sin(Th2)*sin(Th3)*sin(Th4)*sin(Th5)*sin(Th6) - 2.9736e-6*cos(Th2)*cos(Th5)*cos(Th6)^2*sin(Th3)*sin(Th5) - 2.9736e-6*cos(Th3)*cos(Th5)*cos(Th6)^2*sin(Th2)*sin(Th5) + 2.9736e-6*cos(Th2)*cos(Th3)*cos(Th4)*cos(Th5)^2*cos(Th6)^2 - 2.9736e-6*cos(Th4)*cos(Th5)^2*cos(Th6)^2*sin(Th2)*sin(Th3) + 0.000019974*cos(Th2)*cos(Th3)*cos(Th4)*cos(Th5)*cos(Th6)*sin(Th5) - 1.4868e-6*cos(Th2)*cos(Th3)*cos(Th5)*cos(Th6)*sin(Th4)*sin(Th6) - 0.000019974*cos(Th4)*cos(Th5)*cos(Th6)*sin(Th2)*sin(Th3)*sin(Th5) + 1.4868e-6*cos(Th5)*cos(Th6)*sin(Th2)*sin(Th3)*sin(Th4)*sin(Th6))*dTh4*dTh1;
V542=(0.0066904*cos(Th5)^2*sin(Th4) - 0.0033452*sin(Th4) - 1.4868e-6*cos(Th6)^2*sin(Th4) + 6.2e-9*cos(Th4)*cos(Th5) + 0.000019529*cos(Th4)*sin(Th5) + 0.0046569*cos(Th5)*sin(Th4) - 3.8e-6*sin(Th4)*sin(Th5) + 2.9736e-6*cos(Th5)^2*cos(Th6)^2*sin(Th4) + 0.0044118*cos(Th5)*sin(Th3)*sin(Th4) + 6.08e-8*cos(Th5)*sin(Th4)*sin(Th5) + 4.9934e-6*cos(Th4)*sin(Th5)*sin(Th6) + 0.00002185*cos(Th6)*sin(Th4)*sin(Th5) - 3.6e-6*sin(Th3)*sin(Th4)*sin(Th5) + 1.4868e-6*cos(Th4)*cos(Th5)*cos(Th6)*sin(Th6) + 0.000019974*cos(Th5)*cos(Th6)*sin(Th4)*sin(Th5) + 0.0000207*cos(Th6)*sin(Th3)*sin(Th4)*sin(Th5))*dTh4*dTh2;
V543=(6.2e-9*cos(Th4)*cos(Th5) + 0.000019529*cos(Th4)*sin(Th5) + 0.0046569*cos(Th5)*sin(Th4) - 3.8e-6*sin(Th4)*sin(Th5) + 0.003346*sin(Th4)*(2.0*cos(Th5)^2 - 1.0) + 6.08e-8*cos(Th5)*sin(Th4)*sin(Th5) + 4.9934e-6*cos(Th4)*sin(Th5)*sin(Th6) + 0.00002185*cos(Th6)*sin(Th4)*sin(Th5) + 7.4339e-7*sin(Th4)*(2.0*cos(Th5)^2 - 1.0)*(2.0*cos(Th6)^2 - 1.0) + 1.4868e-6*cos(Th4)*cos(Th5)*cos(Th6)*sin(Th6) + 0.000019974*cos(Th5)*cos(Th6)*sin(Th4)*sin(Th5))*dTh4*dTh3;
V544=(6.08e-8*cos(Th5)^2 - 9.9869e-6*cos(Th6) + 0.000019974*cos(Th5)^2*cos(Th6) - 0.0066904*cos(Th5)*sin(Th5) - 2.9736e-6*cos(Th5)*cos(Th6)^2*sin(Th5) - 3.04e-8)*dTh4*dTh4;
V545=(- 6.2e-9*cos(Th5) - 0.000019529*sin(Th5) - 4.9934e-6*sin(Th5)*sin(Th6) - 1.4868e-6*cos(Th5)*cos(Th6)*sin(Th6))*dTh4*dTh5;
V546=(0.000061*sin(Th5) - 1.0*(0.000115*cos(Th6)*sin(Th1)*sin(Th4) - 0.000115*sin(Th2 + Th3)*cos(Th1)*cos(Th4)*cos(Th6) + 0.000115*cos(Th4)*cos(Th5)*sin(Th1)*sin(Th6) + 0.000115*sin(Th2 + Th3)*cos(Th1)*cos(Th5)*sin(Th4)*sin(Th6))*(0.05206*cos(Th2 + Th3)*cos(Th1)*sin(Th5) - 0.05206*cos(Th5)*sin(Th1)*sin(Th4) + 0.05206*sin(Th2 + Th3)*cos(Th1)*cos(Th4)*cos(Th5) - 0.00023*cos(Th6)*sin(Th1)*sin(Th4)*sin(Th5) - 0.00023*cos(Th2 + Th3)*cos(Th1)*cos(Th5)*cos(Th6) + 0.00023*sin(Th2 + Th3)*cos(Th1)*cos(Th4)*cos(Th6)*sin(Th5)) - 6.0e-6*cos(Th6)^2*sin(Th5) + 6.0e-6*cos(Th5)*cos(Th6) + (0.000115*cos(Th1)*cos(Th6)*sin(Th4) + 0.000115*sin(Th2 + Th3)*cos(Th4)*cos(Th6)*sin(Th1) + 0.000115*cos(Th1)*cos(Th4)*cos(Th5)*sin(Th6) - 0.000115*sin(Th2 + Th3)*cos(Th5)*sin(Th1)*sin(Th4)*sin(Th6))*(0.05206*cos(Th2 + Th3)*sin(Th1)*sin(Th5) + 0.05206*cos(Th1)*cos(Th5)*sin(Th4) - 0.00023*cos(Th2 + Th3)*cos(Th5)*cos(Th6)*sin(Th1) + 0.05206*sin(Th2 + Th3)*cos(Th4)*cos(Th5)*sin(Th1) + 0.00023*cos(Th1)*cos(Th6)*sin(Th4)*sin(Th5) + 0.00023*sin(Th2 + Th3)*cos(Th4)*cos(Th6)*sin(Th1)*sin(Th5)) - 0.5*(0.05206*cos(Th5) + 0.00023*cos(Th6)*sin(Th5))*(0.5*cos(Th1)*cos(Th4) - 0.5*sin(Th2 + Th3)*sin(Th1)*sin(Th4))*(0.00023*sin(Th2 + Th3)*cos(Th6)*sin(Th1)*sin(Th4) - 0.00023*cos(Th1)*cos(Th4)*cos(Th6) + 0.00023*cos(Th2 + Th3)*sin(Th1)*sin(Th5)*sin(Th6) + 0.00023*cos(Th1)*cos(Th5)*sin(Th4)*sin(Th6) + 0.00023*sin(Th2 + Th3)*cos(Th4)*cos(Th5)*sin(Th1)*sin(Th6)) + 0.5*cos(Th2 + Th3)*(0.00023*cos(Th4)*cos(Th6) - 0.00023*cos(Th5)*sin(Th4)*sin(Th6))*(0.05206*cos(Th2 + Th3)*cos(Th4)*cos(Th5) - 0.05206*sin(Th2 + Th3)*sin(Th5) + 0.00023*sin(Th2 + Th3)*cos(Th5)*cos(Th6) + 0.00023*cos(Th2 + Th3)*cos(Th4)*cos(Th6)*sin(Th5)) - 0.0000575*sin(Th6)*(cos(Th2 + Th3)*cos(Th1)*cos(Th5) + sin(Th1)*sin(Th4)*sin(Th5) - 1.0*sin(Th2 + Th3)*cos(Th1)*cos(Th4)*sin(Th5))*(0.05206*cos(Th4)*sin(Th1)*sin(Th5) + 0.00023*sin(Th1)*sin(Th4)*sin(Th6) - 0.00023*sin(Th2 + Th3)*cos(Th1)*cos(Th4)*sin(Th6) + 0.05206*sin(Th2 + Th3)*cos(Th1)*sin(Th4)*sin(Th5) - 0.00023*cos(Th4)*cos(Th5)*cos(Th6)*sin(Th1) - 0.00023*sin(Th2 + Th3)*cos(Th1)*cos(Th5)*cos(Th6)*sin(Th4)) - 0.0000575*sin(Th6)*(cos(Th1)*sin(Th4)*sin(Th5) - 1.0*cos(Th2 + Th3)*cos(Th5)*sin(Th1) + sin(Th2 + Th3)*cos(Th4)*sin(Th1)*sin(Th5))*(0.05206*cos(Th1)*cos(Th4)*sin(Th5) + 0.00023*cos(Th1)*sin(Th4)*sin(Th6) + 0.00023*sin(Th2 + Th3)*cos(Th4)*sin(Th1)*sin(Th6) - 0.05206*sin(Th2 + Th3)*sin(Th1)*sin(Th4)*sin(Th5) - 0.00023*cos(Th1)*cos(Th4)*cos(Th5)*cos(Th6) + 0.00023*sin(Th2 + Th3)*cos(Th5)*cos(Th6)*sin(Th1)*sin(Th4)) + 0.5*(0.05206*cos(Th5) + 0.00023*cos(Th6)*sin(Th5))*(cos(Th4)*sin(Th1) + sin(Th2 + Th3)*cos(Th1)*sin(Th4))*(0.000115*cos(Th4)*cos(Th6)*sin(Th1) + 0.000115*sin(Th2 + Th3)*cos(Th1)*cos(Th6)*sin(Th4) + 0.000115*cos(Th2 + Th3)*cos(Th1)*sin(Th5)*sin(Th6) - 0.000115*cos(Th5)*sin(Th1)*sin(Th4)*sin(Th6) + 0.000115*sin(Th2 + Th3)*cos(Th1)*cos(Th4)*cos(Th5)*sin(Th6)) - 0.0000575*cos(Th2 + Th3)*sin(Th6)*(sin(Th2 + Th3)*cos(Th5) + cos(Th2 + Th3)*cos(Th4)*sin(Th5))*(0.00023*cos(Th4)*sin(Th6) - 0.05206*sin(Th4)*sin(Th5) + 0.00023*cos(Th5)*cos(Th6)*sin(Th4)) + 0.25*cos(Th2 + Th3)*sin(Th4)*(0.05206*cos(Th5) + 0.00023*cos(Th6)*sin(Th5))*(0.00023*cos(Th2 + Th3)*cos(Th6)*sin(Th4) - 0.00023*sin(Th2 + Th3)*sin(Th5)*sin(Th6) + 0.00023*cos(Th2 + Th3)*cos(Th4)*cos(Th5)*sin(Th6)))*dTh4*dTh6;
%---------------------------
V551=(6.2e-9*cos(Th2)*cos(Th5)*sin(Th3) - 0.00085785*sin(Th4)*sin(Th5) - 7.0e-7*cos(Th5)*sin(Th4) + 6.2e-9*cos(Th3)*cos(Th5)*sin(Th2) + 4.025e-6*cos(Th5)*cos(Th6)*sin(Th4) + 0.000019529*cos(Th2)*sin(Th3)*sin(Th5) + 0.000019529*cos(Th3)*sin(Th2)*sin(Th5) + 3.6e-6*cos(Th5)*sin(Th2)*sin(Th4) + 0.0044118*sin(Th2)*sin(Th4)*sin(Th5) - 0.000019529*cos(Th2)*cos(Th3)*cos(Th4)*cos(Th5) + 6.2e-9*cos(Th2)*cos(Th3)*cos(Th4)*sin(Th5) - 3.8e-6*cos(Th2)*cos(Th3)*cos(Th5)*sin(Th4) - 0.0046569*cos(Th2)*cos(Th3)*sin(Th4)*sin(Th5) + 0.000019529*cos(Th4)*cos(Th5)*sin(Th2)*sin(Th3) - 0.0000207*cos(Th5)*cos(Th6)*sin(Th2)*sin(Th4) - 6.2e-9*cos(Th4)*sin(Th2)*sin(Th3)*sin(Th5) + 3.8e-6*cos(Th5)*sin(Th2)*sin(Th3)*sin(Th4) + 4.9934e-6*cos(Th2)*sin(Th3)*sin(Th5)*sin(Th6) + 4.9934e-6*cos(Th3)*sin(Th2)*sin(Th5)*sin(Th6) + 0.0046569*sin(Th2)*sin(Th3)*sin(Th4)*sin(Th5) - 4.9934e-6*cos(Th2)*cos(Th3)*cos(Th4)*cos(Th5)*sin(Th6) + 0.00002185*cos(Th2)*cos(Th3)*cos(Th5)*cos(Th6)*sin(Th4) + 1.4868e-6*cos(Th2)*cos(Th5)*cos(Th6)*sin(Th3)*sin(Th6) + 1.4868e-6*cos(Th3)*cos(Th5)*cos(Th6)*sin(Th2)*sin(Th6) + 4.9934e-6*cos(Th4)*cos(Th5)*sin(Th2)*sin(Th3)*sin(Th6) - 0.00002185*cos(Th5)*cos(Th6)*sin(Th2)*sin(Th3)*sin(Th4) + 1.4868e-6*cos(Th2)*cos(Th3)*cos(Th4)*cos(Th6)*sin(Th5)*sin(Th6) - 1.4868e-6*cos(Th4)*cos(Th6)*sin(Th2)*sin(Th3)*sin(Th5)*sin(Th6))*dTh5*dTh1;
V552=(3.8e-6*cos(Th4)*cos(Th5) - 0.0044118*cos(Th3)*cos(Th5) + 3.6e-6*cos(Th3)*sin(Th5) + 0.0046569*cos(Th4)*sin(Th5) - 0.000019529*cos(Th5)*sin(Th4) + 6.2e-9*sin(Th4)*sin(Th5) - 0.00002185*cos(Th4)*cos(Th5)*cos(Th6) + 3.6e-6*cos(Th4)*cos(Th5)*sin(Th3) - 0.0000207*cos(Th3)*cos(Th6)*sin(Th5) + 0.0044118*cos(Th4)*sin(Th3)*sin(Th5) - 4.9934e-6*cos(Th5)*sin(Th4)*sin(Th6) - 0.0000207*cos(Th4)*cos(Th5)*cos(Th6)*sin(Th3) + 1.4868e-6*cos(Th6)*sin(Th4)*sin(Th5)*sin(Th6))*dTh5*dTh2;
V553=(3.8e-6*cos(Th4)*cos(Th5) - 1.0*(0.05206*cos(Th2 + Th3)*sin(Th5) - 0.00023*cos(Th2 + Th3)*cos(Th5)*cos(Th6) + 0.05206*sin(Th2 + Th3)*cos(Th4)*cos(Th5) + 0.00023*sin(Th2 + Th3)*cos(Th4)*cos(Th6)*sin(Th5))*(0.05206*cos(Th2 + Th3)*cos(Th4)*cos(Th5) - 0.05206*sin(Th2 + Th3)*sin(Th5) + 0.00023*sin(Th2 + Th3)*cos(Th5)*cos(Th6) + 0.00023*cos(Th2 + Th3)*cos(Th4)*cos(Th6)*sin(Th5)) - 1.0*(0.00004*sin(Th2 + Th3)*cos(Th5) - 0.00304*sin(Th2 + Th3)*sin(Th5) + 0.00304*cos(Th2 + Th3)*cos(Th4)*cos(Th5) + 0.00004*cos(Th2 + Th3)*cos(Th4)*sin(Th5))*(0.00152*cos(Th2 + Th3)*sin(Th5) - 0.00002*cos(Th2 + Th3)*cos(Th5) + 0.00152*sin(Th2 + Th3)*cos(Th4)*cos(Th5) + 0.00002*sin(Th2 + Th3)*cos(Th4)*sin(Th5)) + 0.0046569*cos(Th4)*sin(Th5) - 0.000019529*cos(Th5)*sin(Th4) + 6.2e-9*sin(Th4)*sin(Th5) + cos(Th1)*(0.05206*cos(Th2 + Th3)*cos(Th4)*cos(Th5) - 0.05206*sin(Th2 + Th3)*sin(Th5) + 0.00023*sin(Th2 + Th3)*cos(Th5)*cos(Th6) + 0.00023*cos(Th2 + Th3)*cos(Th4)*cos(Th6)*sin(Th5))*(0.05206*cos(Th2 + Th3)*cos(Th1)*sin(Th5) - 0.05206*cos(Th5)*sin(Th1)*sin(Th4) + 0.05206*sin(Th2 + Th3)*cos(Th1)*cos(Th4)*cos(Th5) - 0.00023*cos(Th6)*sin(Th1)*sin(Th4)*sin(Th5) - 0.00023*cos(Th2 + Th3)*cos(Th1)*cos(Th5)*cos(Th6) + 0.00023*sin(Th2 + Th3)*cos(Th1)*cos(Th4)*cos(Th6)*sin(Th5)) - 2.0*cos(Th1)*(0.00002*sin(Th2 + Th3)*cos(Th5) - 0.00152*sin(Th2 + Th3)*sin(Th5) + 0.00152*cos(Th2 + Th3)*cos(Th4)*cos(Th5) + 0.00002*cos(Th2 + Th3)*cos(Th4)*sin(Th5))*(0.00002*cos(Th2 + Th3)*cos(Th1)*cos(Th5) - 0.00152*cos(Th2 + Th3)*cos(Th1)*sin(Th5) + 0.00152*cos(Th5)*sin(Th1)*sin(Th4) + 0.00002*sin(Th1)*sin(Th4)*sin(Th5) - 0.00152*sin(Th2 + Th3)*cos(Th1)*cos(Th4)*cos(Th5) - 0.00002*sin(Th2 + Th3)*cos(Th1)*cos(Th4)*sin(Th5)) - 1.3553e-25*sin(Th4)*sin(Th6)*(1.4757e19*cos(Th5) - 1.1068e19*cos(Th6)*sin(Th5)) - 0.00002185*cos(Th4)*cos(Th5)*cos(Th6) - 2.9935e-6*cos(Th5)*sin(Th4)*sin(Th6) + 2.0*sin(Th1)*(0.00002*sin(Th2 + Th3)*cos(Th5) - 0.00152*sin(Th2 + Th3)*sin(Th5) + 0.00152*cos(Th2 + Th3)*cos(Th4)*cos(Th5) + 0.00002*cos(Th2 + Th3)*cos(Th4)*sin(Th5))*(0.00152*cos(Th2 + Th3)*sin(Th1)*sin(Th5) - 0.00002*cos(Th2 + Th3)*cos(Th5)*sin(Th1) + 0.00152*cos(Th1)*cos(Th5)*sin(Th4) + 0.00002*cos(Th1)*sin(Th4)*sin(Th5) + 0.00152*sin(Th2 + Th3)*cos(Th4)*cos(Th5)*sin(Th1) + 0.00002*sin(Th2 + Th3)*cos(Th4)*sin(Th1)*sin(Th5)) + sin(Th1)*(0.05206*cos(Th2 + Th3)*cos(Th4)*cos(Th5) - 0.05206*sin(Th2 + Th3)*sin(Th5) + 0.00023*sin(Th2 + Th3)*cos(Th5)*cos(Th6) + 0.00023*cos(Th2 + Th3)*cos(Th4)*cos(Th6)*sin(Th5))*(0.05206*cos(Th2 + Th3)*sin(Th1)*sin(Th5) + 0.05206*cos(Th1)*cos(Th5)*sin(Th4) - 0.00023*cos(Th2 + Th3)*cos(Th5)*cos(Th6)*sin(Th1) + 0.05206*sin(Th2 + Th3)*cos(Th4)*cos(Th5)*sin(Th1) + 0.00023*cos(Th1)*cos(Th6)*sin(Th4)*sin(Th5) + 0.00023*sin(Th2 + Th3)*cos(Th4)*cos(Th6)*sin(Th1)*sin(Th5)) - 1.3225e-8*cos(Th6)*sin(Th4)*sin(Th5)*sin(Th6))*dTh5*dTh3;
V554=(6.2e-9*cos(Th5) + 0.000019529*sin(Th5) + 4.9934e-6*sin(Th5)*sin(Th6) + 1.4868e-6*cos(Th5)*cos(Th6)*sin(Th6))*dTh5*dTh4;
V555=((0.02603*cos(Th2 + Th3)*cos(Th1)*cos(Th5) + 0.02603*sin(Th1)*sin(Th4)*sin(Th5) + 0.000115*cos(Th2 + Th3)*cos(Th1)*cos(Th6)*sin(Th5) - 0.02603*sin(Th2 + Th3)*cos(Th1)*cos(Th4)*sin(Th5) - 0.000115*cos(Th5)*cos(Th6)*sin(Th1)*sin(Th4) + 0.000115*sin(Th2 + Th3)*cos(Th1)*cos(Th4)*cos(Th5)*cos(Th6))*(0.05206*cos(Th2 + Th3)*cos(Th1)*sin(Th5) - 0.05206*cos(Th5)*sin(Th1)*sin(Th4) + 0.05206*sin(Th2 + Th3)*cos(Th1)*cos(Th4)*cos(Th5) - 0.00023*cos(Th6)*sin(Th1)*sin(Th4)*sin(Th5) - 0.00023*cos(Th2 + Th3)*cos(Th1)*cos(Th5)*cos(Th6) + 0.00023*sin(Th2 + Th3)*cos(Th1)*cos(Th4)*cos(Th6)*sin(Th5)) - 1.0*(0.00002*sin(Th2 + Th3)*cos(Th5) - 0.00152*sin(Th2 + Th3)*sin(Th5) + 0.00152*cos(Th2 + Th3)*cos(Th4)*cos(Th5) + 0.00002*cos(Th2 + Th3)*cos(Th4)*sin(Th5))*(0.00152*sin(Th2 + Th3)*cos(Th5) + 0.00002*sin(Th2 + Th3)*sin(Th5) - 0.00002*cos(Th2 + Th3)*cos(Th4)*cos(Th5) + 0.00152*cos(Th2 + Th3)*cos(Th4)*sin(Th5)) - 1.0*(0.02603*sin(Th2 + Th3)*cos(Th5) + 0.02603*cos(Th2 + Th3)*cos(Th4)*sin(Th5) + 0.000115*sin(Th2 + Th3)*cos(Th6)*sin(Th5) - 0.000115*cos(Th2 + Th3)*cos(Th4)*cos(Th5)*cos(Th6))*(0.05206*cos(Th2 + Th3)*cos(Th4)*cos(Th5) - 0.05206*sin(Th2 + Th3)*sin(Th5) + 0.00023*sin(Th2 + Th3)*cos(Th5)*cos(Th6) + 0.00023*cos(Th2 + Th3)*cos(Th4)*cos(Th6)*sin(Th5)) + (0.02603*cos(Th2 + Th3)*sin(Th1)*sin(Th5) + 0.02603*cos(Th1)*cos(Th5)*sin(Th4) - 0.000115*cos(Th2 + Th3)*cos(Th5)*cos(Th6)*sin(Th1) + 0.02603*sin(Th2 + Th3)*cos(Th4)*cos(Th5)*sin(Th1) + 0.000115*cos(Th1)*cos(Th6)*sin(Th4)*sin(Th5) + 0.000115*sin(Th2 + Th3)*cos(Th4)*cos(Th6)*sin(Th1)*sin(Th5))*(0.05206*cos(Th2 + Th3)*cos(Th5)*sin(Th1) - 0.05206*cos(Th1)*sin(Th4)*sin(Th5) + 0.00023*cos(Th2 + Th3)*cos(Th6)*sin(Th1)*sin(Th5) - 0.05206*sin(Th2 + Th3)*cos(Th4)*sin(Th1)*sin(Th5) + 0.00023*cos(Th1)*cos(Th5)*cos(Th6)*sin(Th4) + 0.00023*sin(Th2 + Th3)*cos(Th4)*cos(Th5)*cos(Th6)*sin(Th1)) + (0.00152*cos(Th2 + Th3)*cos(Th5)*sin(Th1) + 0.00002*cos(Th2 + Th3)*sin(Th1)*sin(Th5) + 0.00002*cos(Th1)*cos(Th5)*sin(Th4) - 0.00152*cos(Th1)*sin(Th4)*sin(Th5) + 0.00002*sin(Th2 + Th3)*cos(Th4)*cos(Th5)*sin(Th1) - 0.00152*sin(Th2 + Th3)*cos(Th4)*sin(Th1)*sin(Th5))*(0.00152*cos(Th2 + Th3)*sin(Th1)*sin(Th5) - 0.00002*cos(Th2 + Th3)*cos(Th5)*sin(Th1) + 0.00152*cos(Th1)*cos(Th5)*sin(Th4) + 0.00002*cos(Th1)*sin(Th4)*sin(Th5) + 0.00152*sin(Th2 + Th3)*cos(Th4)*cos(Th5)*sin(Th1) + 0.00002*sin(Th2 + Th3)*cos(Th4)*sin(Th1)*sin(Th5)) - 1.0*(0.00152*cos(Th2 + Th3)*cos(Th1)*cos(Th5) + 0.00002*cos(Th2 + Th3)*cos(Th1)*sin(Th5) - 0.00002*cos(Th5)*sin(Th1)*sin(Th4) + 0.00152*sin(Th1)*sin(Th4)*sin(Th5) + 0.00002*sin(Th2 + Th3)*cos(Th1)*cos(Th4)*cos(Th5) - 0.00152*sin(Th2 + Th3)*cos(Th1)*cos(Th4)*sin(Th5))*(0.00002*cos(Th2 + Th3)*cos(Th1)*cos(Th5) - 0.00152*cos(Th2 + Th3)*cos(Th1)*sin(Th5) + 0.00152*cos(Th5)*sin(Th1)*sin(Th4) + 0.00002*sin(Th1)*sin(Th4)*sin(Th5) - 0.00152*sin(Th2 + Th3)*cos(Th1)*cos(Th4)*cos(Th5) - 0.00002*sin(Th2 + Th3)*cos(Th1)*cos(Th4)*sin(Th5)))*dTh5*dTh5;
V556=(2.9736e-6*sin(2.0*Th6))*dTh5*dTh6;
%---------------------------
V561=(0.000058013*cos(Th2)*sin(Th3)*sin(Th5) + 0.000058013*cos(Th3)*sin(Th2)*sin(Th5) - 4.025e-6*sin(Th4)*sin(Th5)*sin(Th6) - 0.000058013*cos(Th2)*cos(Th3)*cos(Th4)*cos(Th5) + 4.9934e-6*cos(Th2)*cos(Th5)*cos(Th6)*sin(Th3) + 4.9934e-6*cos(Th3)*cos(Th5)*cos(Th6)*sin(Th2) + 0.000058013*cos(Th4)*cos(Th5)*sin(Th2)*sin(Th3) + 0.0000207*sin(Th2)*sin(Th4)*sin(Th5)*sin(Th6) + 4.9934e-6*cos(Th2)*cos(Th3)*cos(Th4)*cos(Th6)*sin(Th5) - 0.00002185*cos(Th2)*cos(Th3)*sin(Th4)*sin(Th5)*sin(Th6) - 4.9934e-6*cos(Th4)*cos(Th6)*sin(Th2)*sin(Th3)*sin(Th5) + 0.00002185*sin(Th2)*sin(Th3)*sin(Th4)*sin(Th5)*sin(Th6))*dTh6*dTh1;
V562=(0.00002185*cos(Th4)*sin(Th5)*sin(Th6) - 0.0000207*cos(Th3)*cos(Th5)*sin(Th6) - 0.000058013*cos(Th5)*sin(Th4) + 4.9934e-6*cos(Th6)*sin(Th4)*sin(Th5) + 0.0000207*cos(Th4)*sin(Th3)*sin(Th5)*sin(Th6))*dTh6*dTh2;
V563=(0.5*sin(Th1)*(0.00023*cos(Th2 + Th3)*cos(Th6)*sin(Th4) - 0.00023*sin(Th2 + Th3)*sin(Th5)*sin(Th6) + 0.00023*cos(Th2 + Th3)*cos(Th4)*cos(Th5)*sin(Th6))*(0.05206*cos(Th2 + Th3)*sin(Th1)*sin(Th5) + 0.05206*cos(Th1)*cos(Th5)*sin(Th4) - 0.00023*cos(Th2 + Th3)*cos(Th5)*cos(Th6)*sin(Th1) + 0.05206*sin(Th2 + Th3)*cos(Th4)*cos(Th5)*sin(Th1) + 0.00023*cos(Th1)*cos(Th6)*sin(Th4)*sin(Th5) + 0.00023*sin(Th2 + Th3)*cos(Th4)*cos(Th6)*sin(Th1)*sin(Th5)) - 1.0*(0.000115*sin(Th2 + Th3)*cos(Th6)*sin(Th4) + 0.000115*cos(Th2 + Th3)*sin(Th5)*sin(Th6) + 0.000115*sin(Th2 + Th3)*cos(Th4)*cos(Th5)*sin(Th6))*(0.05206*cos(Th2 + Th3)*cos(Th4)*cos(Th5) - 0.05206*sin(Th2 + Th3)*sin(Th5) + 0.00023*sin(Th2 + Th3)*cos(Th5)*cos(Th6) + 0.00023*cos(Th2 + Th3)*cos(Th4)*cos(Th6)*sin(Th5)) - 4.2352e-22*sin(Th4)*(1.3695e17*cos(Th5) - 4.7224e15*cos(Th6)*sin(Th5)) - 1.3225e-8*cos(Th5)*sin(Th4) - 1.0*(0.000115*cos(Th2 + Th3)*cos(Th6)*sin(Th4) - 0.000115*sin(Th2 + Th3)*sin(Th5)*sin(Th6) + 0.000115*cos(Th2 + Th3)*cos(Th4)*cos(Th5)*sin(Th6))*(0.05206*cos(Th2 + Th3)*sin(Th5) - 0.00023*cos(Th2 + Th3)*cos(Th5)*cos(Th6) + 0.05206*sin(Th2 + Th3)*cos(Th4)*cos(Th5) + 0.00023*sin(Th2 + Th3)*cos(Th4)*cos(Th6)*sin(Th5)) + 0.5*cos(Th1)*(0.00023*cos(Th2 + Th3)*cos(Th6)*sin(Th4) - 0.00023*sin(Th2 + Th3)*sin(Th5)*sin(Th6) + 0.00023*cos(Th2 + Th3)*cos(Th4)*cos(Th5)*sin(Th6))*(0.05206*cos(Th2 + Th3)*cos(Th1)*sin(Th5) - 0.05206*cos(Th5)*sin(Th1)*sin(Th4) + 0.05206*sin(Th2 + Th3)*cos(Th1)*cos(Th4)*cos(Th5) - 0.00023*cos(Th6)*sin(Th1)*sin(Th4)*sin(Th5) - 0.00023*cos(Th2 + Th3)*cos(Th1)*cos(Th5)*cos(Th6) + 0.00023*sin(Th2 + Th3)*cos(Th1)*cos(Th4)*cos(Th6)*sin(Th5)) + 0.5*cos(Th1)*(0.05206*cos(Th2 + Th3)*cos(Th4)*cos(Th5) - 0.05206*sin(Th2 + Th3)*sin(Th5) + 0.00023*sin(Th2 + Th3)*cos(Th5)*cos(Th6) + 0.00023*cos(Th2 + Th3)*cos(Th4)*cos(Th6)*sin(Th5))*(0.00023*cos(Th4)*cos(Th6)*sin(Th1) + 0.00023*sin(Th2 + Th3)*cos(Th1)*cos(Th6)*sin(Th4) + 0.00023*cos(Th2 + Th3)*cos(Th1)*sin(Th5)*sin(Th6) - 0.00023*cos(Th5)*sin(Th1)*sin(Th4)*sin(Th6) + 0.00023*sin(Th2 + Th3)*cos(Th1)*cos(Th4)*cos(Th5)*sin(Th6)) + 0.5*sin(Th1)*(0.05206*cos(Th2 + Th3)*cos(Th4)*cos(Th5) - 0.05206*sin(Th2 + Th3)*sin(Th5) + 0.00023*sin(Th2 + Th3)*cos(Th5)*cos(Th6) + 0.00023*cos(Th2 + Th3)*cos(Th4)*cos(Th6)*sin(Th5))*(0.00023*sin(Th2 + Th3)*cos(Th6)*sin(Th1)*sin(Th4) - 0.00023*cos(Th1)*cos(Th4)*cos(Th6) + 0.00023*cos(Th2 + Th3)*sin(Th1)*sin(Th5)*sin(Th6) + 0.00023*cos(Th1)*cos(Th5)*sin(Th4)*sin(Th6) + 0.00023*sin(Th2 + Th3)*cos(Th4)*cos(Th5)*sin(Th1)*sin(Th6)) + 0.00002185*cos(Th4)*sin(Th5)*sin(Th6) + 2.9935e-6*cos(Th6)*sin(Th4)*sin(Th5))*dTh6*dTh3;
V564=(0.000058*sin(Th5) - 1.0*(0.000115*cos(Th6)*sin(Th1)*sin(Th4) - 0.000115*sin(Th2 + Th3)*cos(Th1)*cos(Th4)*cos(Th6) + 0.000115*cos(Th4)*cos(Th5)*sin(Th1)*sin(Th6) + 0.000115*sin(Th2 + Th3)*cos(Th1)*cos(Th5)*sin(Th4)*sin(Th6))*(0.05206*cos(Th2 + Th3)*cos(Th1)*sin(Th5) - 0.05206*cos(Th5)*sin(Th1)*sin(Th4) + 0.05206*sin(Th2 + Th3)*cos(Th1)*cos(Th4)*cos(Th5) - 0.00023*cos(Th6)*sin(Th1)*sin(Th4)*sin(Th5) - 0.00023*cos(Th2 + Th3)*cos(Th1)*cos(Th5)*cos(Th6) + 0.00023*sin(Th2 + Th3)*cos(Th1)*cos(Th4)*cos(Th6)*sin(Th5)) + 2.0e-6*cos(Th5)*cos(Th6) + (0.000115*cos(Th1)*cos(Th6)*sin(Th4) + 0.000115*sin(Th2 + Th3)*cos(Th4)*cos(Th6)*sin(Th1) + 0.000115*cos(Th1)*cos(Th4)*cos(Th5)*sin(Th6) - 0.000115*sin(Th2 + Th3)*cos(Th5)*sin(Th1)*sin(Th4)*sin(Th6))*(0.05206*cos(Th2 + Th3)*sin(Th1)*sin(Th5) + 0.05206*cos(Th1)*cos(Th5)*sin(Th4) - 0.00023*cos(Th2 + Th3)*cos(Th5)*cos(Th6)*sin(Th1) + 0.05206*sin(Th2 + Th3)*cos(Th4)*cos(Th5)*sin(Th1) + 0.00023*cos(Th1)*cos(Th6)*sin(Th4)*sin(Th5) + 0.00023*sin(Th2 + Th3)*cos(Th4)*cos(Th6)*sin(Th1)*sin(Th5)) + 0.5*(0.05206*cos(Th5) + 0.00023*cos(Th6)*sin(Th5))*(0.5*cos(Th1)*cos(Th4) - 0.5*sin(Th2 + Th3)*sin(Th1)*sin(Th4))*(0.00023*sin(Th2 + Th3)*cos(Th6)*sin(Th1)*sin(Th4) - 0.00023*cos(Th1)*cos(Th4)*cos(Th6) + 0.00023*cos(Th2 + Th3)*sin(Th1)*sin(Th5)*sin(Th6) + 0.00023*cos(Th1)*cos(Th5)*sin(Th4)*sin(Th6) + 0.00023*sin(Th2 + Th3)*cos(Th4)*cos(Th5)*sin(Th1)*sin(Th6)) + 0.5*cos(Th2 + Th3)*(0.00023*cos(Th4)*cos(Th6) - 0.00023*cos(Th5)*sin(Th4)*sin(Th6))*(0.05206*cos(Th2 + Th3)*cos(Th4)*cos(Th5) - 0.05206*sin(Th2 + Th3)*sin(Th5) + 0.00023*sin(Th2 + Th3)*cos(Th5)*cos(Th6) + 0.00023*cos(Th2 + Th3)*cos(Th4)*cos(Th6)*sin(Th5)) + 0.0000575*sin(Th6)*(cos(Th2 + Th3)*cos(Th1)*cos(Th5) + sin(Th1)*sin(Th4)*sin(Th5) - 1.0*sin(Th2 + Th3)*cos(Th1)*cos(Th4)*sin(Th5))*(0.05206*cos(Th4)*sin(Th1)*sin(Th5) + 0.00023*sin(Th1)*sin(Th4)*sin(Th6) - 0.00023*sin(Th2 + Th3)*cos(Th1)*cos(Th4)*sin(Th6) + 0.05206*sin(Th2 + Th3)*cos(Th1)*sin(Th4)*sin(Th5) - 0.00023*cos(Th4)*cos(Th5)*cos(Th6)*sin(Th1) - 0.00023*sin(Th2 + Th3)*cos(Th1)*cos(Th5)*cos(Th6)*sin(Th4)) + 0.0000575*sin(Th6)*(cos(Th1)*sin(Th4)*sin(Th5) - 1.0*cos(Th2 + Th3)*cos(Th5)*sin(Th1) + sin(Th2 + Th3)*cos(Th4)*sin(Th1)*sin(Th5))*(0.05206*cos(Th1)*cos(Th4)*sin(Th5) + 0.00023*cos(Th1)*sin(Th4)*sin(Th6) + 0.00023*sin(Th2 + Th3)*cos(Th4)*sin(Th1)*sin(Th6) - 0.05206*sin(Th2 + Th3)*sin(Th1)*sin(Th4)*sin(Th5) - 0.00023*cos(Th1)*cos(Th4)*cos(Th5)*cos(Th6) + 0.00023*sin(Th2 + Th3)*cos(Th5)*cos(Th6)*sin(Th1)*sin(Th4)) - 0.5*(0.05206*cos(Th5) + 0.00023*cos(Th6)*sin(Th5))*(cos(Th4)*sin(Th1) + sin(Th2 + Th3)*cos(Th1)*sin(Th4))*(0.000115*cos(Th4)*cos(Th6)*sin(Th1) + 0.000115*sin(Th2 + Th3)*cos(Th1)*cos(Th6)*sin(Th4) + 0.000115*cos(Th2 + Th3)*cos(Th1)*sin(Th5)*sin(Th6) - 0.000115*cos(Th5)*sin(Th1)*sin(Th4)*sin(Th6) + 0.000115*sin(Th2 + Th3)*cos(Th1)*cos(Th4)*cos(Th5)*sin(Th6)) + 0.0000575*cos(Th2 + Th3)*sin(Th6)*(sin(Th2 + Th3)*cos(Th5) + cos(Th2 + Th3)*cos(Th4)*sin(Th5))*(0.00023*cos(Th4)*sin(Th6) - 0.05206*sin(Th4)*sin(Th5) + 0.00023*cos(Th5)*cos(Th6)*sin(Th4)) - 0.25*cos(Th2 + Th3)*sin(Th4)*(0.05206*cos(Th5) + 0.00023*cos(Th6)*sin(Th5))*(0.00023*cos(Th2 + Th3)*cos(Th6)*sin(Th4) - 0.00023*sin(Th2 + Th3)*sin(Th5)*sin(Th6) + 0.00023*cos(Th2 + Th3)*cos(Th4)*cos(Th5)*sin(Th6)))*dTh6*dTh4;
V565=(0.5*(0.000115*cos(Th4)*cos(Th6)*sin(Th1) + 0.000115*sin(Th2 + Th3)*cos(Th1)*cos(Th6)*sin(Th4) + 0.000115*cos(Th2 + Th3)*cos(Th1)*sin(Th5)*sin(Th6) - 0.000115*cos(Th5)*sin(Th1)*sin(Th4)*sin(Th6) + 0.000115*sin(Th2 + Th3)*cos(Th1)*cos(Th4)*cos(Th5)*sin(Th6))*(0.05206*cos(Th2 + Th3)*cos(Th1)*cos(Th5) + 0.05206*sin(Th1)*sin(Th4)*sin(Th5) + 0.00023*cos(Th2 + Th3)*cos(Th1)*cos(Th6)*sin(Th5) - 0.05206*sin(Th2 + Th3)*cos(Th1)*cos(Th4)*sin(Th5) - 0.00023*cos(Th5)*cos(Th6)*sin(Th1)*sin(Th4) + 0.00023*sin(Th2 + Th3)*cos(Th1)*cos(Th4)*cos(Th5)*cos(Th6)) - 0.5*(0.000115*cos(Th2 + Th3)*cos(Th6)*sin(Th4) - 0.000115*sin(Th2 + Th3)*sin(Th5)*sin(Th6) + 0.000115*cos(Th2 + Th3)*cos(Th4)*cos(Th5)*sin(Th6))*(0.05206*sin(Th2 + Th3)*cos(Th5) + 0.05206*cos(Th2 + Th3)*cos(Th4)*sin(Th5) + 0.00023*sin(Th2 + Th3)*cos(Th6)*sin(Th5) - 0.00023*cos(Th2 + Th3)*cos(Th4)*cos(Th5)*cos(Th6)) + 0.5*(0.000115*sin(Th2 + Th3)*cos(Th6)*sin(Th1)*sin(Th4) - 0.000115*cos(Th1)*cos(Th4)*cos(Th6) + 0.000115*cos(Th2 + Th3)*sin(Th1)*sin(Th5)*sin(Th6) + 0.000115*cos(Th1)*cos(Th5)*sin(Th4)*sin(Th6) + 0.000115*sin(Th2 + Th3)*cos(Th4)*cos(Th5)*sin(Th1)*sin(Th6))*(0.05206*cos(Th2 + Th3)*cos(Th5)*sin(Th1) - 0.05206*cos(Th1)*sin(Th4)*sin(Th5) + 0.00023*cos(Th2 + Th3)*cos(Th6)*sin(Th1)*sin(Th5) - 0.05206*sin(Th2 + Th3)*cos(Th4)*sin(Th1)*sin(Th5) + 0.00023*cos(Th1)*cos(Th5)*cos(Th6)*sin(Th4) + 0.00023*sin(Th2 + Th3)*cos(Th4)*cos(Th5)*cos(Th6)*sin(Th1)) - 0.000115*sin(Th6)*(0.5*sin(Th2 + Th3)*cos(Th5) + 0.5*cos(Th2 + Th3)*cos(Th4)*sin(Th5))*(0.05206*cos(Th2 + Th3)*cos(Th4)*cos(Th5) - 0.05206*sin(Th2 + Th3)*sin(Th5) + 0.00023*sin(Th2 + Th3)*cos(Th5)*cos(Th6) + 0.00023*cos(Th2 + Th3)*cos(Th4)*cos(Th6)*sin(Th5)) - 0.0000575*sin(Th6)*(cos(Th1)*sin(Th4)*sin(Th5) - 1.0*cos(Th2 + Th3)*cos(Th5)*sin(Th1) + sin(Th2 + Th3)*cos(Th4)*sin(Th1)*sin(Th5))*(0.05206*cos(Th2 + Th3)*sin(Th1)*sin(Th5) + 0.05206*cos(Th1)*cos(Th5)*sin(Th4) - 0.00023*cos(Th2 + Th3)*cos(Th5)*cos(Th6)*sin(Th1) + 0.05206*sin(Th2 + Th3)*cos(Th4)*cos(Th5)*sin(Th1) + 0.00023*cos(Th1)*cos(Th6)*sin(Th4)*sin(Th5) + 0.00023*sin(Th2 + Th3)*cos(Th4)*cos(Th6)*sin(Th1)*sin(Th5)) + 0.0000575*sin(Th6)*(cos(Th2 + Th3)*cos(Th1)*cos(Th5) + sin(Th1)*sin(Th4)*sin(Th5) - 1.0*sin(Th2 + Th3)*cos(Th1)*cos(Th4)*sin(Th5))*(0.05206*cos(Th2 + Th3)*cos(Th1)*sin(Th5) - 0.05206*cos(Th5)*sin(Th1)*sin(Th4) + 0.05206*sin(Th2 + Th3)*cos(Th1)*cos(Th4)*cos(Th5) - 0.00023*cos(Th6)*sin(Th1)*sin(Th4)*sin(Th5) - 0.00023*cos(Th2 + Th3)*cos(Th1)*cos(Th5)*cos(Th6) + 0.00023*sin(Th2 + Th3)*cos(Th1)*cos(Th4)*cos(Th6)*sin(Th5)))*dTh6*dTh5;
V566=(4.0e-6*cos(Th6) - 1.0*(0.000115*cos(Th2 + Th3)*sin(Th4)*sin(Th6) + 0.000115*sin(Th2 + Th3)*cos(Th6)*sin(Th5) - 0.000115*cos(Th2 + Th3)*cos(Th4)*cos(Th5)*cos(Th6))*(0.05206*cos(Th2 + Th3)*cos(Th4)*cos(Th5) - 0.05206*sin(Th2 + Th3)*sin(Th5) + 0.00023*sin(Th2 + Th3)*cos(Th5)*cos(Th6) + 0.00023*cos(Th2 + Th3)*cos(Th4)*cos(Th6)*sin(Th5)) + (0.5*(cos(Th2 + Th3)*cos(Th1)*cos(Th5) + sin(Th1)*sin(Th4)*sin(Th5) - 1.0*sin(Th2 + Th3)*cos(Th1)*cos(Th4)*sin(Th5))*(0.00023*cos(Th2 + Th3)*cos(Th6)*sin(Th4) - 0.00023*sin(Th2 + Th3)*sin(Th5)*sin(Th6) + 0.00023*cos(Th2 + Th3)*cos(Th4)*cos(Th5)*sin(Th6)) + 0.5*(0.00023*sin(Th6)*(cos(Th2 + Th3)*cos(Th1)*sin(Th5) - 1.0*cos(Th5)*sin(Th1)*sin(Th4) + sin(Th2 + Th3)*cos(Th1)*cos(Th4)*cos(Th5)) + 0.00023*cos(Th6)*(cos(Th4)*sin(Th1) + sin(Th2 + Th3)*cos(Th1)*sin(Th4)))*(sin(Th2 + Th3)*cos(Th5) + cos(Th2 + Th3)*cos(Th4)*sin(Th5)))*(0.05206*cos(Th2 + Th3)*sin(Th1)*sin(Th5) + 0.05206*cos(Th1)*cos(Th5)*sin(Th4) - 0.00023*cos(Th2 + Th3)*cos(Th5)*cos(Th6)*sin(Th1) + 0.05206*sin(Th2 + Th3)*cos(Th4)*cos(Th5)*sin(Th1) + 0.00023*cos(Th1)*cos(Th6)*sin(Th4)*sin(Th5) + 0.00023*sin(Th2 + Th3)*cos(Th4)*cos(Th6)*sin(Th1)*sin(Th5)) + 1.0*(0.5*(cos(Th1)*sin(Th4)*sin(Th5) - 1.0*cos(Th2 + Th3)*cos(Th5)*sin(Th1) + sin(Th2 + Th3)*cos(Th4)*sin(Th1)*sin(Th5))*(0.00023*cos(Th2 + Th3)*cos(Th6)*sin(Th4) - 0.00023*sin(Th2 + Th3)*sin(Th5)*sin(Th6) + 0.00023*cos(Th2 + Th3)*cos(Th4)*cos(Th5)*sin(Th6)) + 0.5*(sin(Th2 + Th3)*cos(Th5) + cos(Th2 + Th3)*cos(Th4)*sin(Th5))*(0.00023*cos(Th6)*(cos(Th1)*cos(Th4) - 1.0*sin(Th2 + Th3)*sin(Th1)*sin(Th4)) - 0.00023*sin(Th6)*(cos(Th2 + Th3)*sin(Th1)*sin(Th5) + cos(Th1)*cos(Th5)*sin(Th4) + sin(Th2 + Th3)*cos(Th4)*cos(Th5)*sin(Th1))))*(0.05206*cos(Th2 + Th3)*cos(Th1)*sin(Th5) - 0.05206*cos(Th5)*sin(Th1)*sin(Th4) + 0.05206*sin(Th2 + Th3)*cos(Th1)*cos(Th4)*cos(Th5) - 0.00023*cos(Th6)*sin(Th1)*sin(Th4)*sin(Th5) - 0.00023*cos(Th2 + Th3)*cos(Th1)*cos(Th5)*cos(Th6) + 0.00023*sin(Th2 + Th3)*cos(Th1)*cos(Th4)*cos(Th6)*sin(Th5)))*dTh6*dTh6;
%---------------------------
V5 = V511+V512+V513+V514+V515+V516+V521+V522+V523+V524+V525+V526+...
     V531+V532+V533+V534+V535+V536+V541+V542+V543+V544+V545+V546+...
     V551+V552+V553+V554+V555+V556+V561+V562+V563+V564+V565+V566;
end
